simulink model "MainSim"  (R2024a)
settings: Solver=ode4  StartTime=0.0  StopTime=simtime  FixedStep=0.1  RelTol=1e-3
values from neighbouring files (symbols this model uses):
  C = [1 0 0 0 0 0 -1 0 0 0 0 0 ... (45 elements, 5x9)]    [C.mat]
undefined symbols (not defined in the file or in its folder): Ki, Kp, ssest, syys, utrim, xtrim
libraries: neural x680
(part 11 of 12)

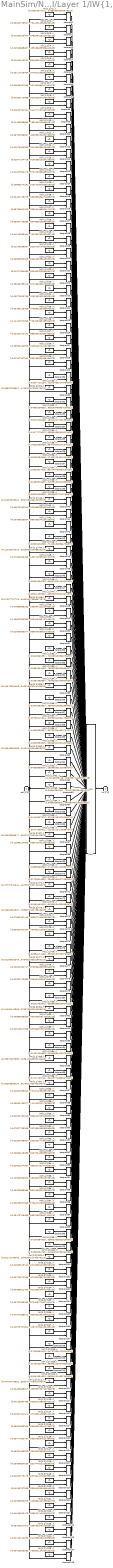
== system MainSim/NARX Neural Network PSI/Layer 1/IW{1,2} ==
  "pd{1,2}" : Inport  PortDimensions=5  SampleTime=0.1
      mask Display: e = 0.06;c1 = [120 230 180]/255;c2 = ([120 230 180]+0)/(256+128);c3 = ([120 230 180]+128)/(256+128);patch([0 1 1 0],[0 0 1 1],c1);patch([0 1 1 1-e 1-e 0+e],[0 0 1 1-e 0+e 0+e],c2);patch([0 0 1 1-e 0+e 0+e],[0 1 1 1-e 1-e 0+e],c3);plot([0 1 1 0 0],[0 0 1 1 0]);
  "IW{1,2}(1,:)'" : Constant  Value=[-0.036215741013831952155310744956295820884406566619873046875;5.60879432784090365695338353813070852993405424058437347412109375e-05;-0.0124726147008203773480783382865411113016307353973388671875;-0.022891343060553341615115385820899973623454570770263671875;0.0202316851446837260575239980653350357897579669952392578125]
      mask Display: e = 0.06;c1 = [120 150 230]/255;c2 = ([120 150 230]+0)/383;c3 = ([120 150 230]+128)/383;patch([0 1 1 0],[0 0 1 1],c1);patch([0 1 1 1-e 1-e 0+e],[0 0 1 1-e 0+e 0+e],c2);patch([0 0 1 1-e 0+e 0+e],[0 1 1 1-e 1-e 0+e],c3);plot([0 1 1 0 0],[0 0 1 1 0]);disp('Weights');
  "IW{1,2}(10,:)'" : Constant  Value=[0.0143353889361894325238377945197498775087296962738037109375;-0.007381001264767226253959986337349619134329259395599365234375;-0.027592123266478564558301656006733537651598453521728515625;0.12178092758731294542595691154929227195680141448974609375;0.1687882806982235195381036874096025712788105010986328125]
      mask Display: e = 0.06;c1 = [120 150 230]/255;c2 = ([120 150 230]+0)/383;c3 = ([120 150 230]+128)/383;patch([0 1 1 0],[0 0 1 1],c1);patch([0 1 1 1-e 1-e 0+e],[0 0 1 1-e 0+e 0+e],c2);patch([0 0 1 1-e 0+e 0+e],[0 1 1 1-e 1-e 0+e],c3);plot([0 1 1 0 0],[0 0 1 1 0]);disp('Weights');
  "IW{1,2}(100,:)'" : Constant  Value=[0.04365501765996560035176798919565044343471527099609375;0.00790203801594095180116372745260377996601164340972900390625;0.01233722257321183228551131350059222313575446605682373046875;-0.036139685759429558686850469939599861390888690948486328125;-0.07424116624505507078257693365230807103216648101806640625]
      mask Display: e = 0.06;c1 = [120 150 230]/255;c2 = ([120 150 230]+0)/383;c3 = ([120 150 230]+128)/383;patch([0 1 1 0],[0 0 1 1],c1);patch([0 1 1 1-e 1-e 0+e],[0 0 1 1-e 0+e 0+e],c2);patch([0 0 1 1-e 0+e 0+e],[0 1 1 1-e 1-e 0+e],c3);plot([0 1 1 0 0],[0 0 1 1 0]);disp('Weights');
  "IW{1,2}(101,:)'" : Constant  Value=[-0.021711480455671894329583437865949235856533050537109375;-0.00807230767060648606026074247665746952407062053680419921875;-0.0002256341632367506698508829998672808869741857051849365234375;-0.0262979277440466806259333765183328068815171718597412109375;-0.011795589954404724075676114125599269755184650421142578125]
      mask Display: e = 0.06;c1 = [120 150 230]/255;c2 = ([120 150 230]+0)/383;c3 = ([120 150 230]+128)/383;patch([0 1 1 0],[0 0 1 1],c1);patch([0 1 1 1-e 1-e 0+e],[0 0 1 1-e 0+e 0+e],c2);patch([0 0 1 1-e 0+e 0+e],[0 1 1 1-e 1-e 0+e],c3);plot([0 1 1 0 0],[0 0 1 1 0]);disp('Weights');
  "IW{1,2}(102,:)'" : Constant  Value=[-0.0190924914203203406615205750540553708560764789581298828125;-0.04084976908135444506608990877793985418975353240966796875;0.01049922442944002665132785523383063264191150665283203125;-0.09276854951829956175135549756305408664047718048095703125;-0.0969975545198410726843718521195114590227603912353515625]
      mask Display: e = 0.06;c1 = [120 150 230]/255;c2 = ([120 150 230]+0)/383;c3 = ([120 150 230]+128)/383;patch([0 1 1 0],[0 0 1 1],c1);patch([0 1 1 1-e 1-e 0+e],[0 0 1 1-e 0+e 0+e],c2);patch([0 0 1 1-e 0+e 0+e],[0 1 1 1-e 1-e 0+e],c3);plot([0 1 1 0 0],[0 0 1 1 0]);disp('Weights');
  "IW{1,2}(103,:)'" : Constant  Value=[-0.037290702881635669208026939713818137533962726593017578125;0.01315953443051502171068367630368811660446226596832275390625;-0.0152059084062875042586693297153033199720084667205810546875;0.011674382342164314751986609053346910513937473297119140625;0.05572879366650791699289158032115665264427661895751953125]
      mask Display: e = 0.06;c1 = [120 150 230]/255;c2 = ([120 150 230]+0)/383;c3 = ([120 150 230]+128)/383;patch([0 1 1 0],[0 0 1 1],c1);patch([0 1 1 1-e 1-e 0+e],[0 0 1 1-e 0+e 0+e],c2);patch([0 0 1 1-e 0+e 0+e],[0 1 1 1-e 1-e 0+e],c3);plot([0 1 1 0 0],[0 0 1 1 0]);disp('Weights');
  "IW{1,2}(104,:)'" : Constant  Value=[-0.00086611442030111451817475654024747200310230255126953125;0.00108653245732205617178622869545279172598384320735931396484375;-0.0300000825214495787929269710048174601979553699493408203125;-0.016134310882040293899652994014104478992521762847900390625;0.044166595105996526993141770844886195845901966094970703125]
      mask Display: e = 0.06;c1 = [120 150 230]/255;c2 = ([120 150 230]+0)/383;c3 = ([120 150 230]+128)/383;patch([0 1 1 0],[0 0 1 1],c1);patch([0 1 1 1-e 1-e 0+e],[0 0 1 1-e 0+e 0+e],c2);patch([0 0 1 1-e 0+e 0+e],[0 1 1 1-e 1-e 0+e],c3);plot([0 1 1 0 0],[0 0 1 1 0]);disp('Weights');
  "IW{1,2}(105,:)'" : Constant  Value=[-0.037679363331454086838423478411641553975641727447509765625;0.02462650060839417787139637994187069125473499298095703125;0.0258598451661068880202964948011867818422615528106689453125;0.06634544811163727018321623063457082025706768035888671875;0.0210341337753423944512132237605328555218875408172607421875]
      mask Display: e = 0.06;c1 = [120 150 230]/255;c2 = ([120 150 230]+0)/383;c3 = ([120 150 230]+128)/383;patch([0 1 1 0],[0 0 1 1],c1);patch([0 1 1 1-e 1-e 0+e],[0 0 1 1-e 0+e 0+e],c2);patch([0 0 1 1-e 0+e 0+e],[0 1 1 1-e 1-e 0+e],c3);plot([0 1 1 0 0],[0 0 1 1 0]);disp('Weights');
  "IW{1,2}(106,:)'" : Constant  Value=[-0.0797208552113842505715268771382397972047328948974609375;-0.004680836346071730151574552536430928739719092845916748046875;0.04106850000033028524892841915061580948531627655029296875;-0.020138888342617448923288492323990794830024242401123046875;-0.0637193215808195823068871277428115718066692352294921875]
      mask Display: e = 0.06;c1 = [120 150 230]/255;c2 = ([120 150 230]+0)/383;c3 = ([120 150 230]+128)/383;patch([0 1 1 0],[0 0 1 1],c1);patch([0 1 1 1-e 1-e 0+e],[0 0 1 1-e 0+e 0+e],c2);patch([0 0 1 1-e 0+e 0+e],[0 1 1 1-e 1-e 0+e],c3);plot([0 1 1 0 0],[0 0 1 1 0]);disp('Weights');
  "IW{1,2}(107,:)'" : Constant  Value=[-0.018787076045366134235958810450028977356851100921630859375;0.038027756628217591894358662329977960325777530670166015625;0.01064586703009156622157238558656899840570986270904541015625;0.043188689285246890936509345237936940975487232208251953125;0.0201443282352079984509618526544727501459419727325439453125]
      mask Display: e = 0.06;c1 = [120 150 230]/255;c2 = ([120 150 230]+0)/383;c3 = ([120 150 230]+128)/383;patch([0 1 1 0],[0 0 1 1],c1);patch([0 1 1 1-e 1-e 0+e],[0 0 1 1-e 0+e 0+e],c2);patch([0 0 1 1-e 0+e 0+e],[0 1 1 1-e 1-e 0+e],c3);plot([0 1 1 0 0],[0 0 1 1 0]);disp('Weights');
  "IW{1,2}(108,:)'" : Constant  Value=[0.07009550418119052384025025048686075024306774139404296875;0.0392247917688698655158674455378786660730838775634765625;-0.06753931344667206404519532725316821597516536712646484375;-0.131338914956515451226692903219372965395450592041015625;-0.01805059031289417414978260012503596954047679901123046875]
      mask Display: e = 0.06;c1 = [120 150 230]/255;c2 = ([120 150 230]+0)/383;c3 = ([120 150 230]+128)/383;patch([0 1 1 0],[0 0 1 1],c1);patch([0 1 1 1-e 1-e 0+e],[0 0 1 1-e 0+e 0+e],c2);patch([0 0 1 1-e 0+e 0+e],[0 1 1 1-e 1-e 0+e],c3);plot([0 1 1 0 0],[0 0 1 1 0]);disp('Weights');
  "IW{1,2}(109,:)'" : Constant  Value=[0.027903264592611394523391510347209987230598926544189453125;-0.018209312551109406441707250223771552555263042449951171875;-0.029560053340425600232332925543232704512774944305419921875;-0.058448597479059671844225931636174209415912628173828125;-0.004503732822406581078056309053181394119746983051300048828125]
      mask Display: e = 0.06;c1 = [120 150 230]/255;c2 = ([120 150 230]+0)/383;c3 = ([120 150 230]+128)/383;patch([0 1 1 0],[0 0 1 1],c1);patch([0 1 1 1-e 1-e 0+e],[0 0 1 1-e 0+e 0+e],c2);patch([0 0 1 1-e 0+e 0+e],[0 1 1 1-e 1-e 0+e],c3);plot([0 1 1 0 0],[0 0 1 1 0]);disp('Weights');
  "IW{1,2}(11,:)'" : Constant  Value=[-0.06784536567335834600367405755605432204902172088623046875;0.057055285864451001087704895553542883135378360748291015625;-0.002680767858079032874007996412046850309707224369049072265625;-0.00491724240786181772400187384164382820017635822296142578125;0.0203640435528099732198636928615087526850402355194091796875]
      mask Display: e = 0.06;c1 = [120 150 230]/255;c2 = ([120 150 230]+0)/383;c3 = ([120 150 230]+128)/383;patch([0 1 1 0],[0 0 1 1],c1);patch([0 1 1 1-e 1-e 0+e],[0 0 1 1-e 0+e 0+e],c2);patch([0 0 1 1-e 0+e 0+e],[0 1 1 1-e 1-e 0+e],c3);plot([0 1 1 0 0],[0 0 1 1 0]);disp('Weights');
  "IW{1,2}(110,:)'" : Constant  Value=[0.0343435492268395758941323947510682046413421630859375;0.01295666519578909069154715183458392857573926448822021484375;0.00708078622384187596205951109595844172872602939605712890625;0.033670595471844887158763270917916088365018367767333984375;0.0003231989567397515147363640242161864080117084085941314697265625]
      mask Display: e = 0.06;c1 = [120 150 230]/255;c2 = ([120 150 230]+0)/383;c3 = ([120 150 230]+128)/383;patch([0 1 1 0],[0 0 1 1],c1);patch([0 1 1 1-e 1-e 0+e],[0 0 1 1-e 0+e 0+e],c2);patch([0 0 1 1-e 0+e 0+e],[0 1 1 1-e 1-e 0+e],c3);plot([0 1 1 0 0],[0 0 1 1 0]);disp('Weights');
  "IW{1,2}(111,:)'" : Constant  Value=[-0.047944793321469260372058585062404745258390903472900390625;0.0476529114527805830459072922167251817882061004638671875;0.024448937097989863198588267323430045507848262786865234375;0.11063606950268144168969541851765825413167476654052734375;0.07017883922331434598529398272148682735860347747802734375]
      mask Display: e = 0.06;c1 = [120 150 230]/255;c2 = ([120 150 230]+0)/383;c3 = ([120 150 230]+128)/383;patch([0 1 1 0],[0 0 1 1],c1);patch([0 1 1 1-e 1-e 0+e],[0 0 1 1-e 0+e 0+e],c2);patch([0 0 1 1-e 0+e 0+e],[0 1 1 1-e 1-e 0+e],c3);plot([0 1 1 0 0],[0 0 1 1 0]);disp('Weights');
  "IW{1,2}(112,:)'" : Constant  Value=[-0.00433683917985687970853003747606635442934930324554443359375;-0.01179886612651101333859582354079975630156695842742919921875;0.038499504319846812594452245548382052220404148101806640625;0.0003384644029183101160244973026891557310591451823711395263671875;-0.07193478992266981453251872835608082823455333709716796875]
      mask Display: e = 0.06;c1 = [120 150 230]/255;c2 = ([120 150 230]+0)/383;c3 = ([120 150 230]+128)/383;patch([0 1 1 0],[0 0 1 1],c1);patch([0 1 1 1-e 1-e 0+e],[0 0 1 1-e 0+e 0+e],c2);patch([0 0 1 1-e 0+e 0+e],[0 1 1 1-e 1-e 0+e],c3);plot([0 1 1 0 0],[0 0 1 1 0]);disp('Weights');
  "IW{1,2}(113,:)'" : Constant  Value=[0.04126094495978659126844689808422117494046688079833984375;0.0715011784149503226704069902552873827517032623291015625;-0.029332417097580047726790297701882082037627696990966796875;0.044113255766767521526272588516803807578980922698974609375;0.0749107750095812374713233339207363314926624298095703125]
      mask Display: e = 0.06;c1 = [120 150 230]/255;c2 = ([120 150 230]+0)/383;c3 = ([120 150 230]+128)/383;patch([0 1 1 0],[0 0 1 1],c1);patch([0 1 1 1-e 1-e 0+e],[0 0 1 1-e 0+e 0+e],c2);patch([0 0 1 1-e 0+e 0+e],[0 1 1 1-e 1-e 0+e],c3);plot([0 1 1 0 0],[0 0 1 1 0]);disp('Weights');
  "IW{1,2}(114,:)'" : Constant  Value=[-0.0156722467499324051576348182379661011509597301483154296875;0.005390025467857165013263465169757182593457400798797607421875;-0.0265373292893429091332535563196870498359203338623046875;0.0001589057175574463335980535116931378070148639380931854248046875;0.056802380327879632704313195290524163283407688140869140625]
      mask Display: e = 0.06;c1 = [120 150 230]/255;c2 = ([120 150 230]+0)/383;c3 = ([120 150 230]+128)/383;patch([0 1 1 0],[0 0 1 1],c1);patch([0 1 1 1-e 1-e 0+e],[0 0 1 1-e 0+e 0+e],c2);patch([0 0 1 1-e 0+e 0+e],[0 1 1 1-e 1-e 0+e],c3);plot([0 1 1 0 0],[0 0 1 1 0]);disp('Weights');
  "IW{1,2}(115,:)'" : Constant  Value=[0.05524953329222011266796954487290349788963794708251953125;-0.006431394135198806143172145510789050604216754436492919921875;-0.062335716365556452511764717883124831132590770721435546875;-0.0139287598417728621102984476465280749835073947906494140625;0.08893091657780860526116839537280611693859100341796875]
      mask Display: e = 0.06;c1 = [120 150 230]/255;c2 = ([120 150 230]+0)/383;c3 = ([120 150 230]+128)/383;patch([0 1 1 0],[0 0 1 1],c1);patch([0 1 1 1-e 1-e 0+e],[0 0 1 1-e 0+e 0+e],c2);patch([0 0 1 1-e 0+e 0+e],[0 1 1 1-e 1-e 0+e],c3);plot([0 1 1 0 0],[0 0 1 1 0]);disp('Weights');
  "IW{1,2}(116,:)'" : Constant  Value=[-0.007770007347034535438723423794726841151714324951171875;0.00179730026795966242765534293113205421832390129566192626953125;-0.0180713848062352931689300561401978484354913234710693359375;-0.0309363499383004843246158799274780903942883014678955078125;0.0110713119878358932923756441368823288939893245697021484375]
      mask Display: e = 0.06;c1 = [120 150 230]/255;c2 = ([120 150 230]+0)/383;c3 = ([120 150 230]+128)/383;patch([0 1 1 0],[0 0 1 1],c1);patch([0 1 1 1-e 1-e 0+e],[0 0 1 1-e 0+e 0+e],c2);patch([0 0 1 1-e 0+e 0+e],[0 1 1 1-e 1-e 0+e],c3);plot([0 1 1 0 0],[0 0 1 1 0]);disp('Weights');
  "IW{1,2}(117,:)'" : Constant  Value=[0.05331469629343903171569962751163984648883342742919921875;-0.00788955748275679651093650335269558127038180828094482421875;-0.041513050258057897223817889198471675626933574676513671875;-0.0931362590739594764510655977574060671031475067138671875;-0.0248034327679624612417175200107521959580481052398681640625]
      mask Display: e = 0.06;c1 = [120 150 230]/255;c2 = ([120 150 230]+0)/383;c3 = ([120 150 230]+128)/383;patch([0 1 1 0],[0 0 1 1],c1);patch([0 1 1 1-e 1-e 0+e],[0 0 1 1-e 0+e 0+e],c2);patch([0 0 1 1-e 0+e 0+e],[0 1 1 1-e 1-e 0+e],c3);plot([0 1 1 0 0],[0 0 1 1 0]);disp('Weights');
  "IW{1,2}(118,:)'" : Constant  Value=[-0.03436657036450664615134797941209399141371250152587890625;-0.0019304738179542059277327137323254646616987884044647216796875;-0.0004147806349897751264886591737734988782904110848903656005859375;-0.05308334180004233016081371943073463626205921173095703125;-0.031944155710130116287981394407324842177331447601318359375]
      mask Display: e = 0.06;c1 = [120 150 230]/255;c2 = ([120 150 230]+0)/383;c3 = ([120 150 230]+128)/383;patch([0 1 1 0],[0 0 1 1],c1);patch([0 1 1 1-e 1-e 0+e],[0 0 1 1-e 0+e 0+e],c2);patch([0 0 1 1-e 0+e 0+e],[0 1 1 1-e 1-e 0+e],c3);plot([0 1 1 0 0],[0 0 1 1 0]);disp('Weights');
  "IW{1,2}(119,:)'" : Constant  Value=[-0.0194977917569244089956992382894895854406058788299560546875;-0.004678634104345880985464933843331891694106161594390869140625;0.05001953115971992380739408190493122674524784088134765625;-0.051358167481461831915812155102685210295021533966064453125;-0.1383571964667627274270245152365532703697681427001953125]
      mask Display: e = 0.06;c1 = [120 150 230]/255;c2 = ([120 150 230]+0)/383;c3 = ([120 150 230]+128)/383;patch([0 1 1 0],[0 0 1 1],c1);patch([0 1 1 1-e 1-e 0+e],[0 0 1 1-e 0+e 0+e],c2);patch([0 0 1 1-e 0+e 0+e],[0 1 1 1-e 1-e 0+e],c3);plot([0 1 1 0 0],[0 0 1 1 0]);disp('Weights');
  "IW{1,2}(12,:)'" : Constant  Value=[-0.016753003332310056894272065619588829576969146728515625;0.0285850979291362959633371332301976508460938930511474609375;0.01179355362913673925528978969623494776897132396697998046875;0.050343408315679884224014273286229581572115421295166015625;0.0247000745497743222356401560091399005614221096038818359375]
      mask Display: e = 0.06;c1 = [120 150 230]/255;c2 = ([120 150 230]+0)/383;c3 = ([120 150 230]+128)/383;patch([0 1 1 0],[0 0 1 1],c1);patch([0 1 1 1-e 1-e 0+e],[0 0 1 1-e 0+e 0+e],c2);patch([0 0 1 1-e 0+e 0+e],[0 1 1 1-e 1-e 0+e],c3);plot([0 1 1 0 0],[0 0 1 1 0]);disp('Weights');
  "IW{1,2}(120,:)'" : Constant  Value=[0.04108767993558308517787480695915292017161846160888671875;0.039495322133149012022723667314494377933442592620849609375;-0.0567553029714990275866881574984290637075901031494140625;-0.0734544757114203861192436306737363338470458984375;0.024152857690850494665202319310992606915533542633056640625]
      mask Display: e = 0.06;c1 = [120 150 230]/255;c2 = ([120 150 230]+0)/383;c3 = ([120 150 230]+128)/383;patch([0 1 1 0],[0 0 1 1],c1);patch([0 1 1 1-e 1-e 0+e],[0 0 1 1-e 0+e 0+e],c2);patch([0 0 1 1-e 0+e 0+e],[0 1 1 1-e 1-e 0+e],c3);plot([0 1 1 0 0],[0 0 1 1 0]);disp('Weights');
  "IW{1,2}(121,:)'" : Constant  Value=[-0.0025880937315550388462537245715111566823907196521759033203125;0.039533967041615707127544254717577132396399974822998046875;-0.0297957396708810710872494809109412017278373241424560546875;0.0175000063548198976637326751415457692928612232208251953125;0.07581829281669293096879158611045568250119686126708984375]
      mask Display: e = 0.06;c1 = [120 150 230]/255;c2 = ([120 150 230]+0)/383;c3 = ([120 150 230]+128)/383;patch([0 1 1 0],[0 0 1 1],c1);patch([0 1 1 1-e 1-e 0+e],[0 0 1 1-e 0+e 0+e],c2);patch([0 0 1 1-e 0+e 0+e],[0 1 1 1-e 1-e 0+e],c3);plot([0 1 1 0 0],[0 0 1 1 0]);disp('Weights');
  "IW{1,2}(122,:)'" : Constant  Value=[-0.040482004756239274578799580694976611994206905364990234375;-0.0084828557419303167452806491155570256523787975311279296875;0.0373609757745712867116338884443393908441066741943359375;0.066359503360522709147772957294364459812641143798828125;0.002060270763875653166063983690037275664508342742919921875]
      mask Display: e = 0.06;c1 = [120 150 230]/255;c2 = ([120 150 230]+0)/383;c3 = ([120 150 230]+128)/383;patch([0 1 1 0],[0 0 1 1],c1);patch([0 1 1 1-e 1-e 0+e],[0 0 1 1-e 0+e 0+e],c2);patch([0 0 1 1-e 0+e 0+e],[0 1 1 1-e 1-e 0+e],c3);plot([0 1 1 0 0],[0 0 1 1 0]);disp('Weights');
  "IW{1,2}(123,:)'" : Constant  Value=[0.03416517870281386703990023079313687048852443695068359375;-0.01497263813686294277316424228274627239443361759185791015625;-0.03330456176119432620819083012975170277059078216552734375;-0.037996513495981439068049922980208066292107105255126953125;0.020667609928990589296393665108553250320255756378173828125]
      mask Display: e = 0.06;c1 = [120 150 230]/255;c2 = ([120 150 230]+0)/383;c3 = ([120 150 230]+128)/383;patch([0 1 1 0],[0 0 1 1],c1);patch([0 1 1 1-e 1-e 0+e],[0 0 1 1-e 0+e 0+e],c2);patch([0 0 1 1-e 0+e 0+e],[0 1 1 1-e 1-e 0+e],c3);plot([0 1 1 0 0],[0 0 1 1 0]);disp('Weights');
  "IW{1,2}(124,:)'" : Constant  Value=[-0.0474311025689617971057288059455459006130695343017578125;-0.0084990343063844515925087108598745544441044330596923828125;0.026522056192171482302821772236711694858968257904052734375;-0.044803604650022366140404983525513671338558197021484375;-0.0706294569851905473800712798038148321211338043212890625]
      mask Display: e = 0.06;c1 = [120 150 230]/255;c2 = ([120 150 230]+0)/383;c3 = ([120 150 230]+128)/383;patch([0 1 1 0],[0 0 1 1],c1);patch([0 1 1 1-e 1-e 0+e],[0 0 1 1-e 0+e 0+e],c2);patch([0 0 1 1-e 0+e 0+e],[0 1 1 1-e 1-e 0+e],c3);plot([0 1 1 0 0],[0 0 1 1 0]);disp('Weights');
  "IW{1,2}(125,:)'" : Constant  Value=[-0.0041352633313304666684562249656664789654314517974853515625;-0.05883224234928326190630087921817903406918048858642578125;0.0446078165266844128833412241874611936509609222412109375;0.10478718971399607340355686346811125986278057098388671875;0.0148238784771977834264777840189708513207733631134033203125]
      mask Display: e = 0.06;c1 = [120 150 230]/255;c2 = ([120 150 230]+0)/383;c3 = ([120 150 230]+128)/383;patch([0 1 1 0],[0 0 1 1],c1);patch([0 1 1 1-e 1-e 0+e],[0 0 1 1-e 0+e 0+e],c2);patch([0 0 1 1-e 0+e 0+e],[0 1 1 1-e 1-e 0+e],c3);plot([0 1 1 0 0],[0 0 1 1 0]);disp('Weights');
  "IW{1,2}(13,:)'" : Constant  Value=[0.02877144728087617508993645287773688323795795440673828125;-0.00416256033542508098455048326513860956765711307525634765625;-0.05354133524824943035635982369058183394372463226318359375;0.06915665582352735485383021796224056743085384368896484375;0.1594088150118338764738012969246483407914638519287109375]
      mask Display: e = 0.06;c1 = [120 150 230]/255;c2 = ([120 150 230]+0)/383;c3 = ([120 150 230]+128)/383;patch([0 1 1 0],[0 0 1 1],c1);patch([0 1 1 1-e 1-e 0+e],[0 0 1 1-e 0+e 0+e],c2);patch([0 0 1 1-e 0+e 0+e],[0 1 1 1-e 1-e 0+e],c3);plot([0 1 1 0 0],[0 0 1 1 0]);disp('Weights');
  "IW{1,2}(14,:)'" : Constant  Value=[-0.04207822478421353873390131639098399318754673004150390625;-0.01012660696863064424544376151970936916768550872802734375;-0.0159495140224796549954788815739448182284832000732421875;0.07987577448249101597088639437060919590294361114501953125;0.12227185354109675052836081476925755850970745086669921875]
      mask Display: e = 0.06;c1 = [120 150 230]/255;c2 = ([120 150 230]+0)/383;c3 = ([120 150 230]+128)/383;patch([0 1 1 0],[0 0 1 1],c1);patch([0 1 1 1-e 1-e 0+e],[0 0 1 1-e 0+e 0+e],c2);patch([0 0 1 1-e 0+e 0+e],[0 1 1 1-e 1-e 0+e],c3);plot([0 1 1 0 0],[0 0 1 1 0]);disp('Weights');
  "IW{1,2}(15,:)'" : Constant  Value=[0.29869274291982061964034755874308757483959197998046875;-0.01021093824654447333732942837514201528392732143402099609375;-0.133787597215125175775796151356189511716365814208984375;-0.172595542507849974978029194971895776689052581787109375;-0.02052316749456706279630680000991560518741607666015625]
      mask Display: e = 0.06;c1 = [120 150 230]/255;c2 = ([120 150 230]+0)/383;c3 = ([120 150 230]+128)/383;patch([0 1 1 0],[0 0 1 1],c1);patch([0 1 1 1-e 1-e 0+e],[0 0 1 1-e 0+e 0+e],c2);patch([0 0 1 1-e 0+e 0+e],[0 1 1 1-e 1-e 0+e],c3);plot([0 1 1 0 0],[0 0 1 1 0]);disp('Weights');
  "IW{1,2}(16,:)'" : Constant  Value=[-0.024547451758043216385463125561727792955935001373291015625;0.0242133921509202522381887234814712428487837314605712890625;-0.0264493059226358594171468752165310434065759181976318359375;-0.0185513623748869392604543548941364861093461513519287109375;0.04532930063992067493128246269407100044190883636474609375]
      mask Display: e = 0.06;c1 = [120 150 230]/255;c2 = ([120 150 230]+0)/383;c3 = ([120 150 230]+128)/383;patch([0 1 1 0],[0 0 1 1],c1);patch([0 1 1 1-e 1-e 0+e],[0 0 1 1-e 0+e 0+e],c2);patch([0 0 1 1-e 0+e 0+e],[0 1 1 1-e 1-e 0+e],c3);plot([0 1 1 0 0],[0 0 1 1 0]);disp('Weights');
  "IW{1,2}(17,:)'" : Constant  Value=[0.05795842020262510774220032772063859738409519195556640625;-0.047212472629454112216240702082359348423779010772705078125;-0.01400780075910705406438960807236071559600532054901123046875;0.08021370444535895483095799818329396657645702362060546875;0.08029121187727565611691460389920393936336040496826171875]
      mask Display: e = 0.06;c1 = [120 150 230]/255;c2 = ([120 150 230]+0)/383;c3 = ([120 150 230]+128)/383;patch([0 1 1 0],[0 0 1 1],c1);patch([0 1 1 1-e 1-e 0+e],[0 0 1 1-e 0+e 0+e],c2);patch([0 0 1 1-e 0+e 0+e],[0 1 1 1-e 1-e 0+e],c3);plot([0 1 1 0 0],[0 0 1 1 0]);disp('Weights');
  "IW{1,2}(18,:)'" : Constant  Value=[-0.0500471888622528171541858910131850279867649078369140625;0.006787486156340967642652817204407256213016808032989501953125;0.053674233914009487900198536181051167659461498260498046875;0.03963848185398781420740732528429361991584300994873046875;-0.0503718037103643434537758594160550273954868316650390625]
      mask Display: e = 0.06;c1 = [120 150 230]/255;c2 = ([120 150 230]+0)/383;c3 = ([120 150 230]+128)/383;patch([0 1 1 0],[0 0 1 1],c1);patch([0 1 1 1-e 1-e 0+e],[0 0 1 1-e 0+e 0+e],c2);patch([0 0 1 1-e 0+e 0+e],[0 1 1 1-e 1-e 0+e],c3);plot([0 1 1 0 0],[0 0 1 1 0]);disp('Weights');
  "IW{1,2}(19,:)'" : Constant  Value=[-0.041135350040979512531436057543032802641391754150390625;0.005798917039239792625693326044711284339427947998046875;-0.01070238640528972141885422075802125618793070316314697265625;-0.0001734097151971002929819742899297807525726966559886932373046875;0.0385962924509451188459507875450071878731250762939453125]
      mask Display: e = 0.06;c1 = [120 150 230]/255;c2 = ([120 150 230]+0)/383;c3 = ([120 150 230]+128)/383;patch([0 1 1 0],[0 0 1 1],c1);patch([0 1 1 1-e 1-e 0+e],[0 0 1 1-e 0+e 0+e],c2);patch([0 0 1 1-e 0+e 0+e],[0 1 1 1-e 1-e 0+e],c3);plot([0 1 1 0 0],[0 0 1 1 0]);disp('Weights');
  "IW{1,2}(2,:)'" : Constant  Value=[-0.0304971550741986729970989244975498877465724945068359375;0.00192189419500140841294555382745556926238350570201873779296875;-0.0179367529279445027390327283001170144416391849517822265625;0.019356188507245401797529638088235515169799327850341796875;0.0644836077260156070867225253095966763794422149658203125]
      mask Display: e = 0.06;c1 = [120 150 230]/255;c2 = ([120 150 230]+0)/383;c3 = ([120 150 230]+128)/383;patch([0 1 1 0],[0 0 1 1],c1);patch([0 1 1 1-e 1-e 0+e],[0 0 1 1-e 0+e 0+e],c2);patch([0 0 1 1-e 0+e 0+e],[0 1 1 1-e 1-e 0+e],c3);plot([0 1 1 0 0],[0 0 1 1 0]);disp('Weights');
  "IW{1,2}(20,:)'" : Constant  Value=[0.01249098007626906793599008693718133145011961460113525390625;-0.007201876217956033714162611403253322350792586803436279296875;0.016084658684607712475500562732122489251196384429931640625;0.04125399740179515328808435015162103809416294097900390625;0.002089202347441310170239603394293226301670074462890625]
      mask Display: e = 0.06;c1 = [120 150 230]/255;c2 = ([120 150 230]+0)/383;c3 = ([120 150 230]+128)/383;patch([0 1 1 0],[0 0 1 1],c1);patch([0 1 1 1-e 1-e 0+e],[0 0 1 1-e 0+e 0+e],c2);patch([0 0 1 1-e 0+e 0+e],[0 1 1 1-e 1-e 0+e],c3);plot([0 1 1 0 0],[0 0 1 1 0]);disp('Weights');
  "IW{1,2}(21,:)'" : Constant  Value=[-0.06392851645465306986704234759599785320460796356201171875;0.0160388436570271901426831817616402986459434032440185546875;0.002192562003192555057651258465512000839225947856903076171875;0.0199696660171350300061465787848646868951618671417236328125;0.038725099380477488730800672556142671965062618255615234375]
      mask Display: e = 0.06;c1 = [120 150 230]/255;c2 = ([120 150 230]+0)/383;c3 = ([120 150 230]+128)/383;patch([0 1 1 0],[0 0 1 1],c1);patch([0 1 1 1-e 1-e 0+e],[0 0 1 1-e 0+e 0+e],c2);patch([0 0 1 1-e 0+e 0+e],[0 1 1 1-e 1-e 0+e],c3);plot([0 1 1 0 0],[0 0 1 1 0]);disp('Weights');
  "IW{1,2}(22,:)'" : Constant  Value=[0.012276845552893787816284287828239030204713344573974609375;0.0088151271711112803852739006060801330022513866424560546875;0.007598114082104707144027511134254382341168820858001708984375;0.0391047021000519856581689737140550278127193450927734375;0.0137905173576384175448961144638815312646329402923583984375]
      mask Display: e = 0.06;c1 = [120 150 230]/255;c2 = ([120 150 230]+0)/383;c3 = ([120 150 230]+128)/383;patch([0 1 1 0],[0 0 1 1],c1);patch([0 1 1 1-e 1-e 0+e],[0 0 1 1-e 0+e 0+e],c2);patch([0 0 1 1-e 0+e 0+e],[0 1 1 1-e 1-e 0+e],c3);plot([0 1 1 0 0],[0 0 1 1 0]);disp('Weights');
  "IW{1,2}(23,:)'" : Constant  Value=[-0.051604951162480483528582908547832630574703216552734375;0.007319954958719951561285643748533402686007320880889892578125;0.062493991229892360828035435815763776190578937530517578125;0.000800132768911692403290825126305207959376275539398193359375;-0.1028039922590014143555237069449503906071186065673828125]
      mask Display: e = 0.06;c1 = [120 150 230]/255;c2 = ([120 150 230]+0)/383;c3 = ([120 150 230]+128)/383;patch([0 1 1 0],[0 0 1 1],c1);patch([0 1 1 1-e 1-e 0+e],[0 0 1 1-e 0+e 0+e],c2);patch([0 0 1 1-e 0+e 0+e],[0 1 1 1-e 1-e 0+e],c3);plot([0 1 1 0 0],[0 0 1 1 0]);disp('Weights');
  "IW{1,2}(24,:)'" : Constant  Value=[-0.032793297385889978723394477810870739631354808807373046875;-0.00725740186413058319114810501559986732900142669677734375;-0.01482374506319721584046700257886186591349542140960693359375;0.01783897550415276811452969241145183332264423370361328125;0.05849075686830969289520254505987395532429218292236328125]
      mask Display: e = 0.06;c1 = [120 150 230]/255;c2 = ([120 150 230]+0)/383;c3 = ([120 150 230]+128)/383;patch([0 1 1 0],[0 0 1 1],c1);patch([0 1 1 1-e 1-e 0+e],[0 0 1 1-e 0+e 0+e],c2);patch([0 0 1 1-e 0+e 0+e],[0 1 1 1-e 1-e 0+e],c3);plot([0 1 1 0 0],[0 0 1 1 0]);disp('Weights');
  "IW{1,2}(25,:)'" : Constant  Value=[-0.06493125428127856368920589602566906251013278961181640625;0.019983209331549518783521790510349092073738574981689453125;0.006643269015488183042161818292470343294553458690643310546875;-0.025892339937117224424323325138175277970731258392333984375;-0.01008616080997910315064647335248082526959478855133056640625]
      mask Display: e = 0.06;c1 = [120 150 230]/255;c2 = ([120 150 230]+0)/383;c3 = ([120 150 230]+128)/383;patch([0 1 1 0],[0 0 1 1],c1);patch([0 1 1 1-e 1-e 0+e],[0 0 1 1-e 0+e 0+e],c2);patch([0 0 1 1-e 0+e 0+e],[0 1 1 1-e 1-e 0+e],c3);plot([0 1 1 0 0],[0 0 1 1 0]);disp('Weights');
  "IW{1,2}(26,:)'" : Constant  Value=[-0.11411371366166600527236596462898887693881988525390625;-0.014919952910250604272146546236399444751441478729248046875;0.035183550637835125929342439121683128178119659423828125;0.049229100632018983618731766682685702107846736907958984375;0.025027472832522372481189876225471380166709423065185546875]
      mask Display: e = 0.06;c1 = [120 150 230]/255;c2 = ([120 150 230]+0)/383;c3 = ([120 150 230]+128)/383;patch([0 1 1 0],[0 0 1 1],c1);patch([0 1 1 1-e 1-e 0+e],[0 0 1 1-e 0+e 0+e],c2);patch([0 0 1 1-e 0+e 0+e],[0 1 1 1-e 1-e 0+e],c3);plot([0 1 1 0 0],[0 0 1 1 0]);disp('Weights');
  "IW{1,2}(27,:)'" : Constant  Value=[-0.0225197214182231535140044087484056944958865642547607421875;0.00736212559279472537887567540337840910069644451141357421875;-0.0135482223952490023199946023169104591943323612213134765625;0.1267734479519667945002225906137027777731418609619140625;0.1598281197241532558539489627946750260889530181884765625]
      mask Display: e = 0.06;c1 = [120 150 230]/255;c2 = ([120 150 230]+0)/383;c3 = ([120 150 230]+128)/383;patch([0 1 1 0],[0 0 1 1],c1);patch([0 1 1 1-e 1-e 0+e],[0 0 1 1-e 0+e 0+e],c2);patch([0 0 1 1-e 0+e 0+e],[0 1 1 1-e 1-e 0+e],c3);plot([0 1 1 0 0],[0 0 1 1 0]);disp('Weights');
  "IW{1,2}(28,:)'" : Constant  Value=[-0.059311625138291905467990972056213649921119213104248046875;-0.006290301789353855595188225180436347727663815021514892578125;0.06314302097769626531675868363890913315117359161376953125;0.05344895511540058430366428865454508922994136810302734375;-0.050575376419835442465267050238253432326018810272216796875]
      mask Display: e = 0.06;c1 = [120 150 230]/255;c2 = ([120 150 230]+0)/383;c3 = ([120 150 230]+128)/383;patch([0 1 1 0],[0 0 1 1],c1);patch([0 1 1 1-e 1-e 0+e],[0 0 1 1-e 0+e 0+e],c2);patch([0 0 1 1-e 0+e 0+e],[0 1 1 1-e 1-e 0+e],c3);plot([0 1 1 0 0],[0 0 1 1 0]);disp('Weights');
  "IW{1,2}(29,:)'" : Constant  Value=[-0.01257287940708441513482096496545636910013854503631591796875;-0.060395065174104041461067282625663210637867450714111328125;0.0491410156741179660055962585829547606408596038818359375;0.11318454423228278826751846963816205970942974090576171875;0.0175407405373560441874669635353711782954633235931396484375]
      mask Display: e = 0.06;c1 = [120 150 230]/255;c2 = ([120 150 230]+0)/383;c3 = ([120 150 230]+128)/383;patch([0 1 1 0],[0 0 1 1],c1);patch([0 1 1 1-e 1-e 0+e],[0 0 1 1-e 0+e 0+e],c2);patch([0 0 1 1-e 0+e 0+e],[0 1 1 1-e 1-e 0+e],c3);plot([0 1 1 0 0],[0 0 1 1 0]);disp('Weights');
  "IW{1,2}(3,:)'" : Constant  Value=[0.01309313474397146882799436440336648956872522830963134765625;-0.0023624846087443381222048532919188801315613090991973876953125;0.03366308921187970149002666175874765031039714813232421875;-0.059173336864796997891513541389940655790269374847412109375;-0.1257206456891222234872884655487723648548126220703125]
      mask Display: e = 0.06;c1 = [120 150 230]/255;c2 = ([120 150 230]+0)/383;c3 = ([120 150 230]+128)/383;patch([0 1 1 0],[0 0 1 1],c1);patch([0 1 1 1-e 1-e 0+e],[0 0 1 1-e 0+e 0+e],c2);patch([0 0 1 1-e 0+e 0+e],[0 1 1 1-e 1-e 0+e],c3);plot([0 1 1 0 0],[0 0 1 1 0]);disp('Weights');
  "IW{1,2}(30,:)'" : Constant  Value=[0.025477231045648675300530072718174778856337070465087890625;-0.00135394366011830683503569527914578429772518575191497802734375;-0.040717708986710905716410735522003960795700550079345703125;-0.03701740728450107764668786103356978856027126312255859375;0.036020242659014455044452773790908395312726497650146484375]
      mask Display: e = 0.06;c1 = [120 150 230]/255;c2 = ([120 150 230]+0)/383;c3 = ([120 150 230]+128)/383;patch([0 1 1 0],[0 0 1 1],c1);patch([0 1 1 1-e 1-e 0+e],[0 0 1 1-e 0+e 0+e],c2);patch([0 0 1 1-e 0+e 0+e],[0 1 1 1-e 1-e 0+e],c3);plot([0 1 1 0 0],[0 0 1 1 0]);disp('Weights');
  "IW{1,2}(31,:)'" : Constant  Value=[-0.08625788597820278902350565886081312783062458038330078125;-0.0015945059916173472298883684317161169019527733325958251953125;0.06342476053783045741862878230676869861781597137451171875;0.10024105858617382569519804746960289776325225830078125;0.0012201089509853405186412533822704062913544476032257080078125]
      mask Display: e = 0.06;c1 = [120 150 230]/255;c2 = ([120 150 230]+0)/383;c3 = ([120 150 230]+128)/383;patch([0 1 1 0],[0 0 1 1],c1);patch([0 1 1 1-e 1-e 0+e],[0 0 1 1-e 0+e 0+e],c2);patch([0 0 1 1-e 0+e 0+e],[0 1 1 1-e 1-e 0+e],c3);plot([0 1 1 0 0],[0 0 1 1 0]);disp('Weights');
  "IW{1,2}(32,:)'" : Constant  Value=[0.0493619805559266655592409733799286186695098876953125;-0.00868653048562638939456004294470403692685067653656005859375;-0.035731840462856878648523206720710732042789459228515625;-0.0809734967866642951772604419602430425584316253662109375;-0.0214995958189504211832687730066027143038809299468994140625]
      mask Display: e = 0.06;c1 = [120 150 230]/255;c2 = ([120 150 230]+0)/383;c3 = ([120 150 230]+128)/383;patch([0 1 1 0],[0 0 1 1],c1);patch([0 1 1 1-e 1-e 0+e],[0 0 1 1-e 0+e 0+e],c2);patch([0 0 1 1-e 0+e 0+e],[0 1 1 1-e 1-e 0+e],c3);plot([0 1 1 0 0],[0 0 1 1 0]);disp('Weights');
  "IW{1,2}(33,:)'" : Constant  Value=[0.00078708469671469002450214791366533972905017435550689697265625;0.01290650907813450411210087764857235015369951725006103515625;0.00046733306145279652522861457697445075609721243381500244140625;0.0818371342885702290903537914346088655292987823486328125;0.07175979228144686861146084311258164234459400177001953125]
      mask Display: e = 0.06;c1 = [120 150 230]/255;c2 = ([120 150 230]+0)/383;c3 = ([120 150 230]+128)/383;patch([0 1 1 0],[0 0 1 1],c1);patch([0 1 1 1-e 1-e 0+e],[0 0 1 1-e 0+e 0+e],c2);patch([0 0 1 1-e 0+e 0+e],[0 1 1 1-e 1-e 0+e],c3);plot([0 1 1 0 0],[0 0 1 1 0]);disp('Weights');
  "IW{1,2}(34,:)'" : Constant  Value=[0.01077275611740714615638392359642239171080291271209716796875;0.00133028746734454423293614322432176777510903775691986083984375;0.0193664306433864973067127124295438989065587520599365234375;0.0107677450955577201641144569066455005668103694915771484375;-0.03386511258580039707144493377199978567659854888916015625]
      mask Display: e = 0.06;c1 = [120 150 230]/255;c2 = ([120 150 230]+0)/383;c3 = ([120 150 230]+128)/383;patch([0 1 1 0],[0 0 1 1],c1);patch([0 1 1 1-e 1-e 0+e],[0 0 1 1-e 0+e 0+e],c2);patch([0 0 1 1-e 0+e 0+e],[0 1 1 1-e 1-e 0+e],c3);plot([0 1 1 0 0],[0 0 1 1 0]);disp('Weights');
  "IW{1,2}(35,:)'" : Constant  Value=[0.18620395058868377535787885790341533720493316650390625;0.0100748286496789123123374309898281353525817394256591796875;-0.098879894409355795215077478133025579154491424560546875;0.01040440551175022231011890738727743155322968959808349609375;0.12380432651178514824596987864424590952694416046142578125]
      mask Display: e = 0.06;c1 = [120 150 230]/255;c2 = ([120 150 230]+0)/383;c3 = ([120 150 230]+128)/383;patch([0 1 1 0],[0 0 1 1],c1);patch([0 1 1 1-e 1-e 0+e],[0 0 1 1-e 0+e 0+e],c2);patch([0 0 1 1-e 0+e 0+e],[0 1 1 1-e 1-e 0+e],c3);plot([0 1 1 0 0],[0 0 1 1 0]);disp('Weights');
  "IW{1,2}(36,:)'" : Constant  Value=[0.06283953308953653393853500119803356938064098358154296875;0.0474044244517978496933352516862214542925357818603515625;-0.03715211937521491203373358302997075952589511871337890625;0.04415491226897565180120608374636503867805004119873046875;0.08324477202418791021987232170431525446474552154541015625]
      mask Display: e = 0.06;c1 = [120 150 230]/255;c2 = ([120 150 230]+0)/383;c3 = ([120 150 230]+128)/383;patch([0 1 1 0],[0 0 1 1],c1);patch([0 1 1 1-e 1-e 0+e],[0 0 1 1-e 0+e 0+e],c2);patch([0 0 1 1-e 0+e 0+e],[0 1 1 1-e 1-e 0+e],c3);plot([0 1 1 0 0],[0 0 1 1 0]);disp('Weights');
  "IW{1,2}(37,:)'" : Constant  Value=[0.10920917616693780194392360272104269824922084808349609375;0.01126622469845997391579839330688628251664340496063232421875;-0.044533761331762129753730761194674414582550525665283203125;-0.0083748004414670833284173312449638615362346172332763671875;0.03457622051458771050835849791837972588837146759033203125]
      mask Display: e = 0.06;c1 = [120 150 230]/255;c2 = ([120 150 230]+0)/383;c3 = ([120 150 230]+128)/383;patch([0 1 1 0],[0 0 1 1],c1);patch([0 1 1 1-e 1-e 0+e],[0 0 1 1-e 0+e 0+e],c2);patch([0 0 1 1-e 0+e 0+e],[0 1 1 1-e 1-e 0+e],c3);plot([0 1 1 0 0],[0 0 1 1 0]);disp('Weights');
  "IW{1,2}(38,:)'" : Constant  Value=[0.01695513639634894931251807292937883175909519195556640625;-0.0025330445163571509679945048532090368098579347133636474609375;-0.040758353940759599332022133921782369725406169891357421875;-0.0020925452959782132010546629174996269284747540950775146484375;0.07235713108715287333883026121839066036045551300048828125]
      mask Display: e = 0.06;c1 = [120 150 230]/255;c2 = ([120 150 230]+0)/383;c3 = ([120 150 230]+128)/383;patch([0 1 1 0],[0 0 1 1],c1);patch([0 1 1 1-e 1-e 0+e],[0 0 1 1-e 0+e 0+e],c2);patch([0 0 1 1-e 0+e 0+e],[0 1 1 1-e 1-e 0+e],c3);plot([0 1 1 0 0],[0 0 1 1 0]);disp('Weights');
  "IW{1,2}(39,:)'" : Constant  Value=[0.060261089685000261695346779333704034797847270965576171875;0.0044640814274999503219465424308509682305157184600830078125;-0.00603114614744149069025525022880174219608306884765625;0.0174924484983870233423264295424814918078482151031494140625;0.00127217357190927550340819873753162028151564300060272216796875]
      mask Display: e = 0.06;c1 = [120 150 230]/255;c2 = ([120 150 230]+0)/383;c3 = ([120 150 230]+128)/383;patch([0 1 1 0],[0 0 1 1],c1);patch([0 1 1 1-e 1-e 0+e],[0 0 1 1-e 0+e 0+e],c2);patch([0 0 1 1-e 0+e 0+e],[0 1 1 1-e 1-e 0+e],c3);plot([0 1 1 0 0],[0 0 1 1 0]);disp('Weights');
  "IW{1,2}(4,:)'" : Constant  Value=[-0.019186886575522539566396318377883289940655231475830078125;-0.004502997689330270718321980183418418164364993572235107421875;0.04010690462661066491012462620346923358738422393798828125;0.03718928157781874188625437227528891526162624359130859375;-0.03608929516841043183550397088765748776495456695556640625]
      mask Display: e = 0.06;c1 = [120 150 230]/255;c2 = ([120 150 230]+0)/383;c3 = ([120 150 230]+128)/383;patch([0 1 1 0],[0 0 1 1],c1);patch([0 1 1 1-e 1-e 0+e],[0 0 1 1-e 0+e 0+e],c2);patch([0 0 1 1-e 0+e 0+e],[0 1 1 1-e 1-e 0+e],c3);plot([0 1 1 0 0],[0 0 1 1 0]);disp('Weights');
  "IW{1,2}(40,:)'" : Constant  Value=[-0.01251919004518711568685329638128678197972476482391357421875;-0.0074290693420022320403450777348552946932613849639892578125;-0.00477620600851305469880525578219021554104983806610107421875;-0.07286144105941876059073791793707641772925853729248046875;-0.0505689571929537340366778153111226856708526611328125]
      mask Display: e = 0.06;c1 = [120 150 230]/255;c2 = ([120 150 230]+0)/383;c3 = ([120 150 230]+128)/383;patch([0 1 1 0],[0 0 1 1],c1);patch([0 1 1 1-e 1-e 0+e],[0 0 1 1-e 0+e 0+e],c2);patch([0 0 1 1-e 0+e 0+e],[0 1 1 1-e 1-e 0+e],c3);plot([0 1 1 0 0],[0 0 1 1 0]);disp('Weights');
  "IW{1,2}(41,:)'" : Constant  Value=[-0.00973192340427684286774390187702010734938085079193115234375;-0.00828568828601327321548009052776251337490975856781005859375;-0.03291887610818965137493563588577671907842159271240234375;0.02531277885914863523542095435914234258234500885009765625;0.0907027874736728023652432284507085569202899932861328125]
      mask Display: e = 0.06;c1 = [120 150 230]/255;c2 = ([120 150 230]+0)/383;c3 = ([120 150 230]+128)/383;patch([0 1 1 0],[0 0 1 1],c1);patch([0 1 1 1-e 1-e 0+e],[0 0 1 1-e 0+e 0+e],c2);patch([0 0 1 1-e 0+e 0+e],[0 1 1 1-e 1-e 0+e],c3);plot([0 1 1 0 0],[0 0 1 1 0]);disp('Weights');
  "IW{1,2}(42,:)'" : Constant  Value=[-0.00795028964429910812994339863735149265266954898834228515625;0.006133615952391663177223346536948156426660716533660888671875;0.012792417644569280266164668091732892207801342010498046875;0.047536670714051799946364695870215655304491519927978515625;0.01857025425068357937785634703686810098588466644287109375]
      mask Display: e = 0.06;c1 = [120 150 230]/255;c2 = ([120 150 230]+0)/383;c3 = ([120 150 230]+128)/383;patch([0 1 1 0],[0 0 1 1],c1);patch([0 1 1 1-e 1-e 0+e],[0 0 1 1-e 0+e 0+e],c2);patch([0 0 1 1-e 0+e 0+e],[0 1 1 1-e 1-e 0+e],c3);plot([0 1 1 0 0],[0 0 1 1 0]);disp('Weights');
  "IW{1,2}(43,:)'" : Constant  Value=[0.00081676808839141966898933500118573647341690957546234130859375;0.0176598623328837640855670798600840498693287372589111328125;0.003015711371351383583705452195999896503053605556488037109375;0.05150230712044646941283332353123114444315433502197265625;0.0369312001607482176535057760702329687774181365966796875]
      mask Display: e = 0.06;c1 = [120 150 230]/255;c2 = ([120 150 230]+0)/383;c3 = ([120 150 230]+128)/383;patch([0 1 1 0],[0 0 1 1],c1);patch([0 1 1 1-e 1-e 0+e],[0 0 1 1-e 0+e 0+e],c2);patch([0 0 1 1-e 0+e 0+e],[0 1 1 1-e 1-e 0+e],c3);plot([0 1 1 0 0],[0 0 1 1 0]);disp('Weights');
  "IW{1,2}(44,:)'" : Constant  Value=[-0.12428194213717647098604857092141173779964447021484375;0.00666044380671207240929287962671878631226718425750732421875;0.0869411568591319794396810038961120881140232086181640625;0.09750588358359453533541483238877844996750354766845703125;-0.03342114122334023662563851075901766307651996612548828125]
      mask Display: e = 0.06;c1 = [120 150 230]/255;c2 = ([120 150 230]+0)/383;c3 = ([120 150 230]+128)/383;patch([0 1 1 0],[0 0 1 1],c1);patch([0 1 1 1-e 1-e 0+e],[0 0 1 1-e 0+e 0+e],c2);patch([0 0 1 1-e 0+e 0+e],[0 1 1 1-e 1-e 0+e],c3);plot([0 1 1 0 0],[0 0 1 1 0]);disp('Weights');
  "IW{1,2}(45,:)'" : Constant  Value=[-0.070816902067406040099939446008647792041301727294921875;0.0164454592017466948161708018005811027251183986663818359375;0.0120979832175336469990423182707672822289168834686279296875;-0.01165481095194141614168614751179120503365993499755859375;-0.006144824907584577056152141949496581219136714935302734375]
      mask Display: e = 0.06;c1 = [120 150 230]/255;c2 = ([120 150 230]+0)/383;c3 = ([120 150 230]+128)/383;patch([0 1 1 0],[0 0 1 1],c1);patch([0 1 1 1-e 1-e 0+e],[0 0 1 1-e 0+e 0+e],c2);patch([0 0 1 1-e 0+e 0+e],[0 1 1 1-e 1-e 0+e],c3);plot([0 1 1 0 0],[0 0 1 1 0]);disp('Weights');
  "IW{1,2}(46,:)'" : Constant  Value=[0.06534094260801122378001792867507901974022388458251953125;-0.0020051330823790364070446923250301551888696849346160888671875;-0.0691351110661047874028639625976211391389369964599609375;0.03938314660646664855381260395006393082439899444580078125;0.1470269811137322746308342402699054218828678131103515625]
      mask Display: e = 0.06;c1 = [120 150 230]/255;c2 = ([120 150 230]+0)/383;c3 = ([120 150 230]+128)/383;patch([0 1 1 0],[0 0 1 1],c1);patch([0 1 1 1-e 1-e 0+e],[0 0 1 1-e 0+e 0+e],c2);patch([0 0 1 1-e 0+e 0+e],[0 1 1 1-e 1-e 0+e],c3);plot([0 1 1 0 0],[0 0 1 1 0]);disp('Weights');
  "IW{1,2}(47,:)'" : Constant  Value=[0.053414398029033451076319494177369051612913608551025390625;-0.0070995937190487558299256676264121779240667819976806640625;0.005288393598413622213871843058541344362311065196990966796875;-0.04910093887565174231024656137378769926726818084716796875;-0.07764435610082069671999960291941533796489238739013671875]
      mask Display: e = 0.06;c1 = [120 150 230]/255;c2 = ([120 150 230]+0)/383;c3 = ([120 150 230]+128)/383;patch([0 1 1 0],[0 0 1 1],c1);patch([0 1 1 1-e 1-e 0+e],[0 0 1 1-e 0+e 0+e],c2);patch([0 0 1 1-e 0+e 0+e],[0 1 1 1-e 1-e 0+e],c3);plot([0 1 1 0 0],[0 0 1 1 0]);disp('Weights');
  "IW{1,2}(48,:)'" : Constant  Value=[-0.0702776772905580049410900755901820957660675048828125;-0.09318722565650006117721204645931720733642578125;0.10187113375325777819835337822951260022819042205810546875;0.107571740968418427808472870310652069747447967529296875;-0.06856554794930551366416437986117671243846416473388671875]
      mask Display: e = 0.06;c1 = [120 150 230]/255;c2 = ([120 150 230]+0)/383;c3 = ([120 150 230]+128)/383;patch([0 1 1 0],[0 0 1 1],c1);patch([0 1 1 1-e 1-e 0+e],[0 0 1 1-e 0+e 0+e],c2);patch([0 0 1 1-e 0+e 0+e],[0 1 1 1-e 1-e 0+e],c3);plot([0 1 1 0 0],[0 0 1 1 0]);disp('Weights');
  "IW{1,2}(49,:)'" : Constant  Value=[-0.0789589526203171576668182751745916903018951416015625;0.0092160245207722028826236027043705689720809459686279296875;0.03332445149348568780300894331958261318504810333251953125;-0.05270797359515333457835595254437066614627838134765625;-0.0815218709533274410450331970423576422035694122314453125]
      mask Display: e = 0.06;c1 = [120 150 230]/255;c2 = ([120 150 230]+0)/383;c3 = ([120 150 230]+128)/383;patch([0 1 1 0],[0 0 1 1],c1);patch([0 1 1 1-e 1-e 0+e],[0 0 1 1-e 0+e 0+e],c2);patch([0 0 1 1-e 0+e 0+e],[0 1 1 1-e 1-e 0+e],c3);plot([0 1 1 0 0],[0 0 1 1 0]);disp('Weights');
  "IW{1,2}(5,:)'" : Constant  Value=[0.010101402217861328580728041970360209234058856964111328125;-0.000614053077992773844138996164332411353825591504573822021484375;0.0195818187383685581026693256490034400485455989837646484375;0.01345489336628006259155565516039132489822804927825927734375;-0.0314055408235604238686988765039131976664066314697265625]
      mask Display: e = 0.06;c1 = [120 150 230]/255;c2 = ([120 150 230]+0)/383;c3 = ([120 150 230]+128)/383;patch([0 1 1 0],[0 0 1 1],c1);patch([0 1 1 1-e 1-e 0+e],[0 0 1 1-e 0+e 0+e],c2);patch([0 0 1 1-e 0+e 0+e],[0 1 1 1-e 1-e 0+e],c3);plot([0 1 1 0 0],[0 0 1 1 0]);disp('Weights');
  "IW{1,2}(50,:)'" : Constant  Value=[-0.19657692983947594456139995600096881389617919921875;0.0292269774182451237687363487793845706619322299957275390625;0.09124215886902618810605503085753298364579677581787109375;0.0166041726280283623295996875413038651458919048309326171875;-0.0846009140168149931238161798319197259843349456787109375]
      mask Display: e = 0.06;c1 = [120 150 230]/255;c2 = ([120 150 230]+0)/383;c3 = ([120 150 230]+128)/383;patch([0 1 1 0],[0 0 1 1],c1);patch([0 1 1 1-e 1-e 0+e],[0 0 1 1-e 0+e 0+e],c2);patch([0 0 1 1-e 0+e 0+e],[0 1 1 1-e 1-e 0+e],c3);plot([0 1 1 0 0],[0 0 1 1 0]);disp('Weights');
  "IW{1,2}(51,:)'" : Constant  Value=[-0.0200553937723044438390385124648673809133470058441162109375;0.005629485509033696315206451998847114737145602703094482421875;0.02691653991382693400513659298667334951460361480712890625;0.032985122986870930861247330767582752741873264312744140625;-0.0175287051223987945525184528605677769519388675689697265625]
      mask Display: e = 0.06;c1 = [120 150 230]/255;c2 = ([120 150 230]+0)/383;c3 = ([120 150 230]+128)/383;patch([0 1 1 0],[0 0 1 1],c1);patch([0 1 1 1-e 1-e 0+e],[0 0 1 1-e 0+e 0+e],c2);patch([0 0 1 1-e 0+e 0+e],[0 1 1 1-e 1-e 0+e],c3);plot([0 1 1 0 0],[0 0 1 1 0]);disp('Weights');
  "IW{1,2}(52,:)'" : Constant  Value=[0.0062086155728596041647460168633188004605472087860107421875;0.00514499081138465770568490853520415839739143848419189453125;0.01282012660580350051076070627686931402422487735748291015625;0.035715536835848125940540143119505955837666988372802734375;0.0028511173621683229099932344041690157609991729259490966796875]
      mask Display: e = 0.06;c1 = [120 150 230]/255;c2 = ([120 150 230]+0)/383;c3 = ([120 150 230]+128)/383;patch([0 1 1 0],[0 0 1 1],c1);patch([0 1 1 1-e 1-e 0+e],[0 0 1 1-e 0+e 0+e],c2);patch([0 0 1 1-e 0+e 0+e],[0 1 1 1-e 1-e 0+e],c3);plot([0 1 1 0 0],[0 0 1 1 0]);disp('Weights');
  "IW{1,2}(53,:)'" : Constant  Value=[0.035625044602090281953277184356920770369470119476318359375;0.009911032735840590024434249016849207691848278045654296875;0.0034697523988826846873256837255894424743019044399261474609375;-0.1373774560376276043793808412374346517026424407958984375;-0.155400431110711334525831261998973786830902099609375]
      mask Display: e = 0.06;c1 = [120 150 230]/255;c2 = ([120 150 230]+0)/383;c3 = ([120 150 230]+128)/383;patch([0 1 1 0],[0 0 1 1],c1);patch([0 1 1 1-e 1-e 0+e],[0 0 1 1-e 0+e 0+e],c2);patch([0 0 1 1-e 0+e 0+e],[0 1 1 1-e 1-e 0+e],c3);plot([0 1 1 0 0],[0 0 1 1 0]);disp('Weights');
  "IW{1,2}(54,:)'" : Constant  Value=[0.0195708586432779829689110329127288423478603363037109375;-0.00785360451670600971663116496301881852559745311737060546875;-0.045976299232901592095590359576817718334496021270751953125;0.0776790687028838799932373149204067885875701904296875;0.157043214364119332326907851893338374793529510498046875]
      mask Display: e = 0.06;c1 = [120 150 230]/255;c2 = ([120 150 230]+0)/383;c3 = ([120 150 230]+128)/383;patch([0 1 1 0],[0 0 1 1],c1);patch([0 1 1 1-e 1-e 0+e],[0 0 1 1-e 0+e 0+e],c2);patch([0 0 1 1-e 0+e 0+e],[0 1 1 1-e 1-e 0+e],c3);plot([0 1 1 0 0],[0 0 1 1 0]);disp('Weights');
  "IW{1,2}(55,:)'" : Constant  Value=[-0.04373920496144718950137786350751412101089954376220703125;0.0088617687558829767724422055152899702079594135284423828125;0.038734451467240797739588487047512899152934551239013671875;0.0663554185015422237636784075220930390059947967529296875;0.00026344708582784850427194189848023597733117640018463134765625]
      mask Display: e = 0.06;c1 = [120 150 230]/255;c2 = ([120 150 230]+0)/383;c3 = ([120 150 230]+128)/383;patch([0 1 1 0],[0 0 1 1],c1);patch([0 1 1 1-e 1-e 0+e],[0 0 1 1-e 0+e 0+e],c2);patch([0 0 1 1-e 0+e 0+e],[0 1 1 1-e 1-e 0+e],c3);plot([0 1 1 0 0],[0 0 1 1 0]);disp('Weights');
  "IW{1,2}(56,:)'" : Constant  Value=[0.029439535675457283170342037692535086534917354583740234375;0.0330578122322633394247759497375227510929107666015625;-0.019233955865888517633432996944975457154214382171630859375;0.049831584308810399075451158523719641380012035369873046875;0.0668206737120435045884647706770920194685459136962890625]
      mask Display: e = 0.06;c1 = [120 150 230]/255;c2 = ([120 150 230]+0)/383;c3 = ([120 150 230]+128)/383;patch([0 1 1 0],[0 0 1 1],c1);patch([0 1 1 1-e 1-e 0+e],[0 0 1 1-e 0+e 0+e],c2);patch([0 0 1 1-e 0+e 0+e],[0 1 1 1-e 1-e 0+e],c3);plot([0 1 1 0 0],[0 0 1 1 0]);disp('Weights');
  "IW{1,2}(57,:)'" : Constant  Value=[0.297532418440825840999508500317460857331752777099609375;-0.034088092708690620469269560999237000942230224609375;-0.14892102986354138760560772425378672778606414794921875;-0.0295061413700503753776427373622937011532485485076904296875;0.1429300612607231346640190849939244799315929412841796875]
      mask Display: e = 0.06;c1 = [120 150 230]/255;c2 = ([120 150 230]+0)/383;c3 = ([120 150 230]+128)/383;patch([0 1 1 0],[0 0 1 1],c1);patch([0 1 1 1-e 1-e 0+e],[0 0 1 1-e 0+e 0+e],c2);patch([0 0 1 1-e 0+e 0+e],[0 1 1 1-e 1-e 0+e],c3);plot([0 1 1 0 0],[0 0 1 1 0]);disp('Weights');
  "IW{1,2}(58,:)'" : Constant  Value=[0.046050588079049416256882665265948162414133548736572265625;-0.004610178140486079732818236465163863613270223140716552734375;-0.005728020777426158505196696069106110371649265289306640625;0.0489876732144139681590644386233179830014705657958984375;0.03693442596369800323685694820596836507320404052734375]
      mask Display: e = 0.06;c1 = [120 150 230]/255;c2 = ([120 150 230]+0)/383;c3 = ([120 150 230]+128)/383;patch([0 1 1 0],[0 0 1 1],c1);patch([0 1 1 1-e 1-e 0+e],[0 0 1 1-e 0+e 0+e],c2);patch([0 0 1 1-e 0+e 0+e],[0 1 1 1-e 1-e 0+e],c3);plot([0 1 1 0 0],[0 0 1 1 0]);disp('Weights');
  "IW{1,2}(59,:)'" : Constant  Value=[0.103009398151029163415159928263165056705474853515625;-0.0121680562744036456501728338253087713383138179779052734375;-0.07828735455464851111795354654532275162637233734130859375;-0.05780213635912208325340344572396134026348590850830078125;0.062596398520664620068743033698410727083683013916015625]
      mask Display: e = 0.06;c1 = [120 150 230]/255;c2 = ([120 150 230]+0)/383;c3 = ([120 150 230]+128)/383;patch([0 1 1 0],[0 0 1 1],c1);patch([0 1 1 1-e 1-e 0+e],[0 0 1 1-e 0+e 0+e],c2);patch([0 0 1 1-e 0+e 0+e],[0 1 1 1-e 1-e 0+e],c3);plot([0 1 1 0 0],[0 0 1 1 0]);disp('Weights');
  "IW{1,2}(6,:)'" : Constant  Value=[-0.0311791890698206904108946702081084367819130420684814453125;0.016995459719213755478417482436270802281796932220458984375;0.03188624420348902532840185131135513074696063995361328125;0.060422817949356659450454998250279459170997142791748046875;0.0030955897049768075525444377404937768005765974521636962890625]
      mask Display: e = 0.06;c1 = [120 150 230]/255;c2 = ([120 150 230]+0)/383;c3 = ([120 150 230]+128)/383;patch([0 1 1 0],[0 0 1 1],c1);patch([0 1 1 1-e 1-e 0+e],[0 0 1 1-e 0+e 0+e],c2);patch([0 0 1 1-e 0+e 0+e],[0 1 1 1-e 1-e 0+e],c3);plot([0 1 1 0 0],[0 0 1 1 0]);disp('Weights');
  "IW{1,2}(60,:)'" : Constant  Value=[-0.053186640687095491919489376186902518384158611297607421875;0.011134950294196067910323932892424636520445346832275390625;0.00869066832351204909823394473278312943875789642333984375;-0.043615569086009491062139176165146636776626110076904296875;-0.035103731099999264941846632837041397579014301300048828125]
      mask Display: e = 0.06;c1 = [120 150 230]/255;c2 = ([120 150 230]+0)/383;c3 = ([120 150 230]+128)/383;patch([0 1 1 0],[0 0 1 1],c1);patch([0 1 1 1-e 1-e 0+e],[0 0 1 1-e 0+e 0+e],c2);patch([0 0 1 1-e 0+e 0+e],[0 1 1 1-e 1-e 0+e],c3);plot([0 1 1 0 0],[0 0 1 1 0]);disp('Weights');
  "IW{1,2}(61,:)'" : Constant  Value=[0.04383895007263693965882112024701200425624847412109375;-0.00417775384777785245560277616050370852462947368621826171875;-0.05562356096120750492683981747177313081920146942138671875;-0.01632167143483632953948614385808468796312808990478515625;0.07791084271427604901472108167581609450280666351318359375]
      mask Display: e = 0.06;c1 = [120 150 230]/255;c2 = ([120 150 230]+0)/383;c3 = ([120 150 230]+128)/383;patch([0 1 1 0],[0 0 1 1],c1);patch([0 1 1 1-e 1-e 0+e],[0 0 1 1-e 0+e 0+e],c2);patch([0 0 1 1-e 0+e 0+e],[0 1 1 1-e 1-e 0+e],c3);plot([0 1 1 0 0],[0 0 1 1 0]);disp('Weights');
  "IW{1,2}(62,:)'" : Constant  Value=[-0.01163205148010725518969987746231709024868905544281005859375;0.005786232476052026452162380110166850499808788299560546875;0.0302453572830208954058672787823525140993297100067138671875;0.022926763495360942546330562663570162840187549591064453125;-0.035530279260345874747795136272543459199368953704833984375]
      mask Display: e = 0.06;c1 = [120 150 230]/255;c2 = ([120 150 230]+0)/383;c3 = ([120 150 230]+128)/383;patch([0 1 1 0],[0 0 1 1],c1);patch([0 1 1 1-e 1-e 0+e],[0 0 1 1-e 0+e 0+e],c2);patch([0 0 1 1-e 0+e 0+e],[0 1 1 1-e 1-e 0+e],c3);plot([0 1 1 0 0],[0 0 1 1 0]);disp('Weights');
  "IW{1,2}(63,:)'" : Constant  Value=[0.03548355233459417334973551305665750987827777862548828125;0.010527872219217644655930854469261248596012592315673828125;-0.011956914718693513466352129626102396287024021148681640625;0.030182421685183889736858731112079112790524959564208984375;0.03336747753743972422224572937921038828790187835693359375]
      mask Display: e = 0.06;c1 = [120 150 230]/255;c2 = ([120 150 230]+0)/383;c3 = ([120 150 230]+128)/383;patch([0 1 1 0],[0 0 1 1],c1);patch([0 1 1 1-e 1-e 0+e],[0 0 1 1-e 0+e 0+e],c2);patch([0 0 1 1-e 0+e 0+e],[0 1 1 1-e 1-e 0+e],c3);plot([0 1 1 0 0],[0 0 1 1 0]);disp('Weights');
  "IW{1,2}(64,:)'" : Constant  Value=[0.056500688265350491878979966031693038530647754669189453125;-0.0096651946281269170146988045644320663996040821075439453125;-0.044878679492911043025227257885489962063729763031005859375;-0.0646623951386925688300522097051725722849369049072265625;0.0091006982208810573153900946863359422422945499420166015625]
      mask Display: e = 0.06;c1 = [120 150 230]/255;c2 = ([120 150 230]+0)/383;c3 = ([120 150 230]+128)/383;patch([0 1 1 0],[0 0 1 1],c1);patch([0 1 1 1-e 1-e 0+e],[0 0 1 1-e 0+e 0+e],c2);patch([0 0 1 1-e 0+e 0+e],[0 1 1 1-e 1-e 0+e],c3);plot([0 1 1 0 0],[0 0 1 1 0]);disp('Weights');
  "IW{1,2}(65,:)'" : Constant  Value=[0.01416907376275116682562416059454335481859743595123291015625;0.0028483949521762781144362808305459111579693853855133056640625;0.0308722162659755931801708328521272051148116588592529296875;-0.04724337387927927955910689661322976462543010711669921875;-0.10979134175569719988896366658082115463912487030029296875]
      mask Display: e = 0.06;c1 = [120 150 230]/255;c2 = ([120 150 230]+0)/383;c3 = ([120 150 230]+128)/383;patch([0 1 1 0],[0 0 1 1],c1);patch([0 1 1 1-e 1-e 0+e],[0 0 1 1-e 0+e 0+e],c2);patch([0 0 1 1-e 0+e 0+e],[0 1 1 1-e 1-e 0+e],c3);plot([0 1 1 0 0],[0 0 1 1 0]);disp('Weights');
  "IW{1,2}(66,:)'" : Constant  Value=[0.037478006113766525186914435607832274399697780609130859375;-0.0280962849206550062397536038361067767255008220672607421875;0.00728610926092497675210513108368104440160095691680908203125;0.062707864274675007010273475316353142261505126953125;0.02898778434853831187378858658121316693723201751708984375]
      mask Display: e = 0.06;c1 = [120 150 230]/255;c2 = ([120 150 230]+0)/383;c3 = ([120 150 230]+128)/383;patch([0 1 1 0],[0 0 1 1],c1);patch([0 1 1 1-e 1-e 0+e],[0 0 1 1-e 0+e 0+e],c2);patch([0 0 1 1-e 0+e 0+e],[0 1 1 1-e 1-e 0+e],c3);plot([0 1 1 0 0],[0 0 1 1 0]);disp('Weights');
  "IW{1,2}(67,:)'" : Constant  Value=[-0.00623989977413751985280132572597722173668444156646728515625;0.0059009639551497634901711109023381141014397144317626953125;0.0334060075036575476747913171493564732372760772705078125;-0.003173055203902507004354305308879702351987361907958984375;-0.0674116744791228017508188941064872778952121734619140625]
      mask Display: e = 0.06;c1 = [120 150 230]/255;c2 = ([120 150 230]+0)/383;c3 = ([120 150 230]+128)/383;patch([0 1 1 0],[0 0 1 1],c1);patch([0 1 1 1-e 1-e 0+e],[0 0 1 1-e 0+e 0+e],c2);patch([0 0 1 1-e 0+e 0+e],[0 1 1 1-e 1-e 0+e],c3);plot([0 1 1 0 0],[0 0 1 1 0]);disp('Weights');
  "IW{1,2}(68,:)'" : Constant  Value=[-0.1285611480379074966773345067849732004106044769287109375;0.016943883999349783342491804205565131269395351409912109375;0.0850319704032116707725919013682869262993335723876953125;0.1059187758975919935178211517268209718167781829833984375;-0.0207655887558300146500389615766835049726068973541259765625]
      mask Display: e = 0.06;c1 = [120 150 230]/255;c2 = ([120 150 230]+0)/383;c3 = ([120 150 230]+128)/383;patch([0 1 1 0],[0 0 1 1],c1);patch([0 1 1 1-e 1-e 0+e],[0 0 1 1-e 0+e 0+e],c2);patch([0 0 1 1-e 0+e 0+e],[0 1 1 1-e 1-e 0+e],c3);plot([0 1 1 0 0],[0 0 1 1 0]);disp('Weights');
  "IW{1,2}(69,:)'" : Constant  Value=[0.168830699282009166761753249375033192336559295654296875;0.0359064220121265431640011911440524272620677947998046875;-0.082979500299221464754140242803259752690792083740234375;0.024969373544354224458974300659974687732756137847900390625;0.11331437167191658887954730516867130063474178314208984375]
      mask Display: e = 0.06;c1 = [120 150 230]/255;c2 = ([120 150 230]+0)/383;c3 = ([120 150 230]+128)/383;patch([0 1 1 0],[0 0 1 1],c1);patch([0 1 1 1-e 1-e 0+e],[0 0 1 1-e 0+e 0+e],c2);patch([0 0 1 1-e 0+e 0+e],[0 1 1 1-e 1-e 0+e],c3);plot([0 1 1 0 0],[0 0 1 1 0]);disp('Weights');
  "IW{1,2}(7,:)'" : Constant  Value=[-0.006280376853883662402466825369629077613353729248046875;-0.006448412693169601299369997349231198313646018505096435546875;-0.0202966079096140901427691716207846184261143207550048828125;-0.06175054801947814364648792206935468129813671112060546875;-0.0118466026803576811310403371635402436368167400360107421875]
      mask Display: e = 0.06;c1 = [120 150 230]/255;c2 = ([120 150 230]+0)/383;c3 = ([120 150 230]+128)/383;patch([0 1 1 0],[0 0 1 1],c1);patch([0 1 1 1-e 1-e 0+e],[0 0 1 1-e 0+e 0+e],c2);patch([0 0 1 1-e 0+e 0+e],[0 1 1 1-e 1-e 0+e],c3);plot([0 1 1 0 0],[0 0 1 1 0]);disp('Weights');
  "IW{1,2}(70,:)'" : Constant  Value=[0.02709614692098034904876868722567451186478137969970703125;-0.00906562667680456922558729360162033117376267910003662109375;-0.0203103458889562528411065756017706007696688175201416015625;-0.0708029415983756627017697837800369597971439361572265625;-0.03293545988036851446256747522056684829294681549072265625]
      mask Display: e = 0.06;c1 = [120 150 230]/255;c2 = ([120 150 230]+0)/383;c3 = ([120 150 230]+128)/383;patch([0 1 1 0],[0 0 1 1],c1);patch([0 1 1 1-e 1-e 0+e],[0 0 1 1-e 0+e 0+e],c2);patch([0 0 1 1-e 0+e 0+e],[0 1 1 1-e 1-e 0+e],c3);plot([0 1 1 0 0],[0 0 1 1 0]);disp('Weights');
  "IW{1,2}(71,:)'" : Constant  Value=[-0.1272734264441099105713561812081024982035160064697265625;0.01044732934238230825929605316559900529682636260986328125;0.049855817292208594315727765433621243573725223541259765625;0.170428366146471221842517707045772112905979156494140625;0.11685818113976141618959303514202474616467952728271484375]
      mask Display: e = 0.06;c1 = [120 150 230]/255;c2 = ([120 150 230]+0)/383;c3 = ([120 150 230]+128)/383;patch([0 1 1 0],[0 0 1 1],c1);patch([0 1 1 1-e 1-e 0+e],[0 0 1 1-e 0+e 0+e],c2);patch([0 0 1 1-e 0+e 0+e],[0 1 1 1-e 1-e 0+e],c3);plot([0 1 1 0 0],[0 0 1 1 0]);disp('Weights');
  "IW{1,2}(72,:)'" : Constant  Value=[0.01484401515593502217382759766906019649468362331390380859375;0.03218399273867970922236025899110245518386363983154296875;-0.002979484916718726228435087932666647247970104217529296875;0.067947213431189645849173075475846417248249053955078125;0.058928439543882070450475652023669681511819362640380859375]
      mask Display: e = 0.06;c1 = [120 150 230]/255;c2 = ([120 150 230]+0)/383;c3 = ([120 150 230]+128)/383;patch([0 1 1 0],[0 0 1 1],c1);patch([0 1 1 1-e 1-e 0+e],[0 0 1 1-e 0+e 0+e],c2);patch([0 0 1 1-e 0+e 0+e],[0 1 1 1-e 1-e 0+e],c3);plot([0 1 1 0 0],[0 0 1 1 0]);disp('Weights');
  "IW{1,2}(73,:)'" : Constant  Value=[-0.00662354827651624213091796633534613647498190402984619140625;-0.03330948348265920511135362858112785033881664276123046875;-0.0031173124861200236963842957749193374183960258960723876953125;-0.077467741809885526382828402347513474524021148681640625;-0.060641361550719898032557608757997513748705387115478515625]
      mask Display: e = 0.06;c1 = [120 150 230]/255;c2 = ([120 150 230]+0)/383;c3 = ([120 150 230]+128)/383;patch([0 1 1 0],[0 0 1 1],c1);patch([0 1 1 1-e 1-e 0+e],[0 0 1 1-e 0+e 0+e],c2);patch([0 0 1 1-e 0+e 0+e],[0 1 1 1-e 1-e 0+e],c3);plot([0 1 1 0 0],[0 0 1 1 0]);disp('Weights');
  "IW{1,2}(74,:)'" : Constant  Value=[-0.0765226744550026871660719507417525164783000946044921875;-0.0629949108643587940559172011489863507449626922607421875;0.0269826229678792606225812278353259898722171783447265625;-0.07232021250449793825509914313443005084991455078125;-0.08774125893122229624676577941499999724328517913818359375]
      mask Display: e = 0.06;c1 = [120 150 230]/255;c2 = ([120 150 230]+0)/383;c3 = ([120 150 230]+128)/383;patch([0 1 1 0],[0 0 1 1],c1);patch([0 1 1 1-e 1-e 0+e],[0 0 1 1-e 0+e 0+e],c2);patch([0 0 1 1-e 0+e 0+e],[0 1 1 1-e 1-e 0+e],c3);plot([0 1 1 0 0],[0 0 1 1 0]);disp('Weights');
  "IW{1,2}(75,:)'" : Constant  Value=[-0.05002424034769416272272479773164377547800540924072265625;-0.012413810162381681834187219237719546072185039520263671875;0.0392216032563809380295793971527018584311008453369140625;0.07817232206270242900192357637934037484228610992431640625;0.013632157583722957772121020525446510873734951019287109375]
      mask Display: e = 0.06;c1 = [120 150 230]/255;c2 = ([120 150 230]+0)/383;c3 = ([120 150 230]+128)/383;patch([0 1 1 0],[0 0 1 1],c1);patch([0 1 1 1-e 1-e 0+e],[0 0 1 1-e 0+e 0+e],c2);patch([0 0 1 1-e 0+e 0+e],[0 1 1 1-e 1-e 0+e],c3);plot([0 1 1 0 0],[0 0 1 1 0]);disp('Weights');
  "IW{1,2}(76,:)'" : Constant  Value=[0.0298647443345664322100763143907897756434977054595947265625;-0.02763319342700609748675333321443758904933929443359375;-0.01544331563243443554422906771605994435958564281463623046875;-0.07936006184212930636423521946198889054358005523681640625;-0.05050877487341998151038069408969022333621978759765625]
      mask Display: e = 0.06;c1 = [120 150 230]/255;c2 = ([120 150 230]+0)/383;c3 = ([120 150 230]+128)/383;patch([0 1 1 0],[0 0 1 1],c1);patch([0 1 1 1-e 1-e 0+e],[0 0 1 1-e 0+e 0+e],c2);patch([0 0 1 1-e 0+e 0+e],[0 1 1 1-e 1-e 0+e],c3);plot([0 1 1 0 0],[0 0 1 1 0]);disp('Weights');
  "IW{1,2}(77,:)'" : Constant  Value=[-0.01169332349246907619411128820274825557135045528411865234375;0.1443364276033036464053083136604982428252696990966796875;-0.04952655687030636799672578263198374770581722259521484375;0.0249240366059819036526068458670124527998268604278564453125;0.11632002061284037186528195206847158260643482208251953125]
      mask Display: e = 0.06;c1 = [120 150 230]/255;c2 = ([120 150 230]+0)/383;c3 = ([120 150 230]+128)/383;patch([0 1 1 0],[0 0 1 1],c1);patch([0 1 1 1-e 1-e 0+e],[0 0 1 1-e 0+e 0+e],c2);patch([0 0 1 1-e 0+e 0+e],[0 1 1 1-e 1-e 0+e],c3);plot([0 1 1 0 0],[0 0 1 1 0]);disp('Weights');
  "IW{1,2}(78,:)'" : Constant  Value=[-0.0020125174748483166085877282824867506860755383968353271484375;0.03190546428362150965796217860770411789417266845703125;-0.004882234453004231401751500385444160201586782932281494140625;0.1497948535376275314145999573156586848199367523193359375;0.1596592009022403668705436530217411927878856658935546875]
      mask Display: e = 0.06;c1 = [120 150 230]/255;c2 = ([120 150 230]+0)/383;c3 = ([120 150 230]+128)/383;patch([0 1 1 0],[0 0 1 1],c1);patch([0 1 1 1-e 1-e 0+e],[0 0 1 1-e 0+e 0+e],c2);patch([0 0 1 1-e 0+e 0+e],[0 1 1 1-e 1-e 0+e],c3);plot([0 1 1 0 0],[0 0 1 1 0]);disp('Weights');
  "IW{1,2}(79,:)'" : Constant  Value=[-0.0228717565017696779217093450142783694900572299957275390625;0.001759787609959452374386312811793686705641448497772216796875;-0.0252986868881747810344773341739710303954780101776123046875;0.0307986727002874383085639919954701326787471771240234375;0.0863401148481389990596568395631038583815097808837890625]
      mask Display: e = 0.06;c1 = [120 150 230]/255;c2 = ([120 150 230]+0)/383;c3 = ([120 150 230]+128)/383;patch([0 1 1 0],[0 0 1 1],c1);patch([0 1 1 1-e 1-e 0+e],[0 0 1 1-e 0+e 0+e],c2);patch([0 0 1 1-e 0+e 0+e],[0 1 1 1-e 1-e 0+e],c3);plot([0 1 1 0 0],[0 0 1 1 0]);disp('Weights');
  "IW{1,2}(8,:)'" : Constant  Value=[0.046367108880403858084395807281907764263451099395751953125;0.00168542206739497242053149594909200459369458258152008056640625;0.01183222638417159335022521560176755883730947971343994140625;-0.0664061407782430002111340172632480971515178680419921875;-0.10325489235921285480213072105470928363502025604248046875]
      mask Display: e = 0.06;c1 = [120 150 230]/255;c2 = ([120 150 230]+0)/383;c3 = ([120 150 230]+128)/383;patch([0 1 1 0],[0 0 1 1],c1);patch([0 1 1 1-e 1-e 0+e],[0 0 1 1-e 0+e 0+e],c2);patch([0 0 1 1-e 0+e 0+e],[0 1 1 1-e 1-e 0+e],c3);plot([0 1 1 0 0],[0 0 1 1 0]);disp('Weights');
  "IW{1,2}(80,:)'" : Constant  Value=[0.00242433973091161526769443668172243633307516574859619140625;-0.0084130955172444059353420442448623361997306346893310546875;0.01336072432992155799291733586642294540069997310638427734375;0.063182555118927063997347204349352978169918060302734375;0.0307155057896809254025516366937154089100658893585205078125]
      mask Display: e = 0.06;c1 = [120 150 230]/255;c2 = ([120 150 230]+0)/383;c3 = ([120 150 230]+128)/383;patch([0 1 1 0],[0 0 1 1],c1);patch([0 1 1 1-e 1-e 0+e],[0 0 1 1-e 0+e 0+e],c2);patch([0 0 1 1-e 0+e 0+e],[0 1 1 1-e 1-e 0+e],c3);plot([0 1 1 0 0],[0 0 1 1 0]);disp('Weights');
  "IW{1,2}(81,:)'" : Constant  Value=[-0.041904425666155951935021306553608155809342861175537109375;0.00658958792671388536577037342567564337514340877532958984375;0.03552023322501186852750976186143816448748111724853515625;-0.1151146335386567243208588706693262793123722076416015625;-0.168513629193430436448153386663761921226978302001953125]
      mask Display: e = 0.06;c1 = [120 150 230]/255;c2 = ([120 150 230]+0)/383;c3 = ([120 150 230]+128)/383;patch([0 1 1 0],[0 0 1 1],c1);patch([0 1 1 1-e 1-e 0+e],[0 0 1 1-e 0+e 0+e],c2);patch([0 0 1 1-e 0+e 0+e],[0 1 1 1-e 1-e 0+e],c3);plot([0 1 1 0 0],[0 0 1 1 0]);disp('Weights');
  "IW{1,2}(82,:)'" : Constant  Value=[-0.00889638500304427808085261375481422874145209789276123046875;0.00324502319811211491218383429213645285926759243011474609375;-0.0311693975373349592417060449633936514146625995635986328125;0.0204825654171228201116949918514364981092512607574462890625;0.08338868488624584518476012817700393497943878173828125]
      mask Display: e = 0.06;c1 = [120 150 230]/255;c2 = ([120 150 230]+0)/383;c3 = ([120 150 230]+128)/383;patch([0 1 1 0],[0 0 1 1],c1);patch([0 1 1 1-e 1-e 0+e],[0 0 1 1-e 0+e 0+e],c2);patch([0 0 1 1-e 0+e 0+e],[0 1 1 1-e 1-e 0+e],c3);plot([0 1 1 0 0],[0 0 1 1 0]);disp('Weights');
  "IW{1,2}(83,:)'" : Constant  Value=[-0.01676547506257063113732641568276449106633663177490234375;0.0087035631759373177640526364484685473144054412841796875;-0.01056046042669889391263371436480156262405216693878173828125;-0.066715153697562257217867909275810234248638153076171875;-0.032808911994657748156800636252228287048637866973876953125]
      mask Display: e = 0.06;c1 = [120 150 230]/255;c2 = ([120 150 230]+0)/383;c3 = ([120 150 230]+128)/383;patch([0 1 1 0],[0 0 1 1],c1);patch([0 1 1 1-e 1-e 0+e],[0 0 1 1-e 0+e 0+e],c2);patch([0 0 1 1-e 0+e 0+e],[0 1 1 1-e 1-e 0+e],c3);plot([0 1 1 0 0],[0 0 1 1 0]);disp('Weights');
  "IW{1,2}(84,:)'" : Constant  Value=[0.0123130098307969275406303921727158012799918651580810546875;0.0028049269645423970283293346739128537592478096485137939453125;0.00824660145692025954577974999892830965109169483184814453125;0.0722092022054929838503767314250580966472625732421875;0.04357217270310827228474437333716196008026599884033203125]
      mask Display: e = 0.06;c1 = [120 150 230]/255;c2 = ([120 150 230]+0)/383;c3 = ([120 150 230]+128)/383;patch([0 1 1 0],[0 0 1 1],c1);patch([0 1 1 1-e 1-e 0+e],[0 0 1 1-e 0+e 0+e],c2);patch([0 0 1 1-e 0+e 0+e],[0 1 1 1-e 1-e 0+e],c3);plot([0 1 1 0 0],[0 0 1 1 0]);disp('Weights');
  "IW{1,2}(85,:)'" : Constant  Value=[-0.038722078893211213379554891389489057473838329315185546875;0.001744540471324718990120405948118786909617483615875244140625;-0.0172082590616888277124107986537637771107256412506103515625;0.036617758892380190827164909705970785580575466156005859375;0.0819038563665162033800015706219710409641265869140625]
      mask Display: e = 0.06;c1 = [120 150 230]/255;c2 = ([120 150 230]+0)/383;c3 = ([120 150 230]+128)/383;patch([0 1 1 0],[0 0 1 1],c1);patch([0 1 1 1-e 1-e 0+e],[0 0 1 1-e 0+e 0+e],c2);patch([0 0 1 1-e 0+e 0+e],[0 1 1 1-e 1-e 0+e],c3);plot([0 1 1 0 0],[0 0 1 1 0]);disp('Weights');
  "IW{1,2}(86,:)'" : Constant  Value=[0.047117637426651516607822856030907132662832736968994140625;-0.028827455596412303318043512945223483256995677947998046875;0.00550958456487406385282401544145614025183022022247314453125;-0.0512290298363665963510271694758557714521884918212890625;-0.07661456142018625847800450401337002404034137725830078125]
      mask Display: e = 0.06;c1 = [120 150 230]/255;c2 = ([120 150 230]+0)/383;c3 = ([120 150 230]+128)/383;patch([0 1 1 0],[0 0 1 1],c1);patch([0 1 1 1-e 1-e 0+e],[0 0 1 1-e 0+e 0+e],c2);patch([0 0 1 1-e 0+e 0+e],[0 1 1 1-e 1-e 0+e],c3);plot([0 1 1 0 0],[0 0 1 1 0]);disp('Weights');
  "IW{1,2}(87,:)'" : Constant  Value=[-0.0020655813471467938773062922308554334449581801891326904296875;0.00776598610027402248834338394090082147158682346343994140625;0.01439942258983055445309418018950964324176311492919921875;0.044821573730011103620096690747232059948146343231201171875;0.01110380335180936005323726334381717606447637081146240234375]
      mask Display: e = 0.06;c1 = [120 150 230]/255;c2 = ([120 150 230]+0)/383;c3 = ([120 150 230]+128)/383;patch([0 1 1 0],[0 0 1 1],c1);patch([0 1 1 1-e 1-e 0+e],[0 0 1 1-e 0+e 0+e],c2);patch([0 0 1 1-e 0+e 0+e],[0 1 1 1-e 1-e 0+e],c3);plot([0 1 1 0 0],[0 0 1 1 0]);disp('Weights');
  "IW{1,2}(88,:)'" : Constant  Value=[-0.0160733094294609468732915047439746558666229248046875;0.00090557772402789890771324099461025980417616665363311767578125;0.03446369187478293127924189320765435695648193359375;0.02109689649226643981538842353984364308416843414306640625;-0.043419023846199673866141921507733059115707874298095703125]
      mask Display: e = 0.06;c1 = [120 150 230]/255;c2 = ([120 150 230]+0)/383;c3 = ([120 150 230]+128)/383;patch([0 1 1 0],[0 0 1 1],c1);patch([0 1 1 1-e 1-e 0+e],[0 0 1 1-e 0+e 0+e],c2);patch([0 0 1 1-e 0+e 0+e],[0 1 1 1-e 1-e 0+e],c3);plot([0 1 1 0 0],[0 0 1 1 0]);disp('Weights');
  "IW{1,2}(89,:)'" : Constant  Value=[-0.03500763577537240045511879316109116189181804656982421875;-0.001634813641418610651034892811139798141084611415863037109375;-0.018839114131199700963303911294133285991847515106201171875;0.08585685954516643347833593225004733540117740631103515625;0.131350736620477082094993193095433525741100311279296875]
      mask Display: e = 0.06;c1 = [120 150 230]/255;c2 = ([120 150 230]+0)/383;c3 = ([120 150 230]+128)/383;patch([0 1 1 0],[0 0 1 1],c1);patch([0 1 1 1-e 1-e 0+e],[0 0 1 1-e 0+e 0+e],c2);patch([0 0 1 1-e 0+e 0+e],[0 1 1 1-e 1-e 0+e],c3);plot([0 1 1 0 0],[0 0 1 1 0]);disp('Weights');
  "IW{1,2}(9,:)'" : Constant  Value=[-0.0484976420463635593538498369525768794119358062744140625;-0.00339367449206574335607289327754187979735434055328369140625;0.01252502066403327236898679331034145434387028217315673828125;-0.052184635040541549333426019074977375566959381103515625;-0.051245774833881395371459888110621250234544277191162109375]
      mask Display: e = 0.06;c1 = [120 150 230]/255;c2 = ([120 150 230]+0)/383;c3 = ([120 150 230]+128)/383;patch([0 1 1 0],[0 0 1 1],c1);patch([0 1 1 1-e 1-e 0+e],[0 0 1 1-e 0+e 0+e],c2);patch([0 0 1 1-e 0+e 0+e],[0 1 1 1-e 1-e 0+e],c3);plot([0 1 1 0 0],[0 0 1 1 0]);disp('Weights');
  "IW{1,2}(90,:)'" : Constant  Value=[-0.0109176261920139218430936267623110325075685977935791015625;0.0288048532074580802830876535836068796925246715545654296875;0.00981009956273464801823624981125249178148806095123291015625;0.073950472324662841483444708501338027417659759521484375;0.050421857216715236515991449550710967741906642913818359375]
      mask Display: e = 0.06;c1 = [120 150 230]/255;c2 = ([120 150 230]+0)/383;c3 = ([120 150 230]+128)/383;patch([0 1 1 0],[0 0 1 1],c1);patch([0 1 1 1-e 1-e 0+e],[0 0 1 1-e 0+e 0+e],c2);patch([0 0 1 1-e 0+e 0+e],[0 1 1 1-e 1-e 0+e],c3);plot([0 1 1 0 0],[0 0 1 1 0]);disp('Weights');
  "IW{1,2}(91,:)'" : Constant  Value=[-0.07827795306876676739715747999071027152240276336669921875;-0.007125604461579477556798511983515709289349615573883056640625;0.044951549018300514248824839569351752288639545440673828125;-0.087301579693083664057695614246767945587635040283203125;-0.145779803851686262650133585339062847197055816650390625]
      mask Display: e = 0.06;c1 = [120 150 230]/255;c2 = ([120 150 230]+0)/383;c3 = ([120 150 230]+128)/383;patch([0 1 1 0],[0 0 1 1],c1);patch([0 1 1 1-e 1-e 0+e],[0 0 1 1-e 0+e 0+e],c2);patch([0 0 1 1-e 0+e 0+e],[0 1 1 1-e 1-e 0+e],c3);plot([0 1 1 0 0],[0 0 1 1 0]);disp('Weights');
  "IW{1,2}(92,:)'" : Constant  Value=[-0.0233443560700996068091317425796660245396196842193603515625;-0.01965661959004581793575283654718077741563320159912109375;0.038956501539266837064179327398960595019161701202392578125;0.0666932513252659064928451471132575534284114837646484375;-0.00443994214356853607317265897336255875416100025177001953125]
      mask Display: e = 0.06;c1 = [120 150 230]/255;c2 = ([120 150 230]+0)/383;c3 = ([120 150 230]+128)/383;patch([0 1 1 0],[0 0 1 1],c1);patch([0 1 1 1-e 1-e 0+e],[0 0 1 1-e 0+e 0+e],c2);patch([0 0 1 1-e 0+e 0+e],[0 1 1 1-e 1-e 0+e],c3);plot([0 1 1 0 0],[0 0 1 1 0]);disp('Weights');
  "IW{1,2}(93,:)'" : Constant  Value=[-0.0280614865884632226633588203412728034891188144683837890625;0.0101067236352357751882902192619440029375255107879638671875;0.040459119539689593347819851487656706012785434722900390625;0.019032632102801587403728689196213963441550731658935546875;-0.05312932529971307882288300561413052491843700408935546875]
      mask Display: e = 0.06;c1 = [120 150 230]/255;c2 = ([120 150 230]+0)/383;c3 = ([120 150 230]+128)/383;patch([0 1 1 0],[0 0 1 1],c1);patch([0 1 1 1-e 1-e 0+e],[0 0 1 1-e 0+e 0+e],c2);patch([0 0 1 1-e 0+e 0+e],[0 1 1 1-e 1-e 0+e],c3);plot([0 1 1 0 0],[0 0 1 1 0]);disp('Weights');
  "IW{1,2}(94,:)'" : Constant  Value=[-0.0180237435453893431180905082555909757502377033233642578125;-0.00149831599683425431036865038691985319019295275211334228515625;-0.005911199091877290291707769398499294766224920749664306640625;-0.023213413815095083891915095364311127923429012298583984375;-0.0033078482348178768999991117283343555754981935024261474609375]
      mask Display: e = 0.06;c1 = [120 150 230]/255;c2 = ([120 150 230]+0)/383;c3 = ([120 150 230]+128)/383;patch([0 1 1 0],[0 0 1 1],c1);patch([0 1 1 1-e 1-e 0+e],[0 0 1 1-e 0+e 0+e],c2);patch([0 0 1 1-e 0+e 0+e],[0 1 1 1-e 1-e 0+e],c3);plot([0 1 1 0 0],[0 0 1 1 0]);disp('Weights');
  "IW{1,2}(95,:)'" : Constant  Value=[-0.1298459062237030947617455467479885555803775787353515625;0.05535958711240472618353436473626061342656612396240234375;0.054034599075738924678358188202764722518622875213623046875;0.164507728636724748216835223502130247652530670166015625;0.10315145429831747148075038467140984721481800079345703125]
      mask Display: e = 0.06;c1 = [120 150 230]/255;c2 = ([120 150 230]+0)/383;c3 = ([120 150 230]+128)/383;patch([0 1 1 0],[0 0 1 1],c1);patch([0 1 1 1-e 1-e 0+e],[0 0 1 1-e 0+e 0+e],c2);patch([0 0 1 1-e 0+e 0+e],[0 1 1 1-e 1-e 0+e],c3);plot([0 1 1 0 0],[0 0 1 1 0]);disp('Weights');
  "IW{1,2}(96,:)'" : Constant  Value=[-0.002908889833235703097080726564627184416167438030242919921875;0.044609472269952023248951178402421646751463413238525390625;0.00999226594835701809049766097814426757395267486572265625;0.1342387674244666373457590680118300952017307281494140625;0.10872887514901850847248709897030494175851345062255859375]
      mask Display: e = 0.06;c1 = [120 150 230]/255;c2 = ([120 150 230]+0)/383;c3 = ([120 150 230]+128)/383;patch([0 1 1 0],[0 0 1 1],c1);patch([0 1 1 1-e 1-e 0+e],[0 0 1 1-e 0+e 0+e],c2);patch([0 0 1 1-e 0+e 0+e],[0 1 1 1-e 1-e 0+e],c3);plot([0 1 1 0 0],[0 0 1 1 0]);disp('Weights');
  "IW{1,2}(97,:)'" : Constant  Value=[-0.030185176680019236428176299114056746475398540496826171875;-0.0021777377495732544963880084054608232690952718257904052734375;-0.0017585751410032321624676843185852703754790127277374267578125;-0.0137349325040490473359700018818330136127769947052001953125;0.005187639615479648115548005904429373913444578647613525390625]
      mask Display: e = 0.06;c1 = [120 150 230]/255;c2 = ([120 150 230]+0)/383;c3 = ([120 150 230]+128)/383;patch([0 1 1 0],[0 0 1 1],c1);patch([0 1 1 1-e 1-e 0+e],[0 0 1 1-e 0+e 0+e],c2);patch([0 0 1 1-e 0+e 0+e],[0 1 1 1-e 1-e 0+e],c3);plot([0 1 1 0 0],[0 0 1 1 0]);disp('Weights');
  "IW{1,2}(98,:)'" : Constant  Value=[-0.054757069687668080693043748397030867636203765869140625;0.015329329474747556416591720562792033888399600982666015625;0.047266643743484597350867915110939065925776958465576171875;0.0415885492312116078483796854925458319485187530517578125;-0.036417128879369480010108617307196254841983318328857421875]
      mask Display: e = 0.06;c1 = [120 150 230]/255;c2 = ([120 150 230]+0)/383;c3 = ([120 150 230]+128)/383;patch([0 1 1 0],[0 0 1 1],c1);patch([0 1 1 1-e 1-e 0+e],[0 0 1 1-e 0+e 0+e],c2);patch([0 0 1 1-e 0+e 0+e],[0 1 1 1-e 1-e 0+e],c3);plot([0 1 1 0 0],[0 0 1 1 0]);disp('Weights');
  "IW{1,2}(99,:)'" : Constant  Value=[0.041943843354097794240420427058779750950634479522705078125;0.046909351896642102752732483850195421837270259857177734375;-0.021381639625762616230275625639478676021099090576171875;0.045995326965924621109849113054224289953708648681640625;0.06251407402016632974817156309654819779098033905029296875]
      mask Display: e = 0.06;c1 = [120 150 230]/255;c2 = ([120 150 230]+0)/383;c3 = ([120 150 230]+128)/383;patch([0 1 1 0],[0 0 1 1],c1);patch([0 1 1 1-e 1-e 0+e],[0 0 1 1-e 0+e 0+e],c2);patch([0 0 1 1-e 0+e 0+e],[0 1 1 1-e 1-e 0+e],c3);plot([0 1 1 0 0],[0 0 1 1 0]);disp('Weights');
  Mux : Mux  Inputs=125
      mask Display: e = 0.06;c1 = [120 150 230]/255;c2 = ([120 150 230]+0)/383;c3 = ([120 150 230]+128)/383;patch([0 1 1 0],[0 0 1 1],c1);patch([0 1 1 1-e 1-e 0+e],[0 0 1 1-e 0+e 0+e],c2);patch([0 0 1 1-e 0+e 0+e],[0 1 1 1-e 1-e 0+e],c3);plot([0 1 1 0 0],[0 0 1 1 0]);disp('Mux');
  dotprod{1..125} (125 alike) : neural/Weight Functions/dotprod
  "iz{1,2}" : Outport
      mask Display: e = 0.06;c1 = [120 230 180]/255;c2 = ([120 230 180]+0)/(256+128);c3 = ([120 230 180]+128)/(256+128);patch([0 1 1 0],[0 0 1 1],c1);patch([0 1 1 1-e 1-e 0+e],[0 0 1 1-e 0+e 0+e],c2);patch([0 0 1 1-e 0+e 0+e],[0 1 1 1-e 1-e 0+e],c3);plot([0 1 1 0 0],[0 0 1 1 0]);
  wires:
  Mux/1 -> "iz{1,2}"/1
  dotprod125/1 -> Mux/125
  "IW{1,2}(125,:)'"/1 -> dotprod125/1
  dotprod124/1 -> Mux/124
  "IW{1,2}(124,:)'"/1 -> dotprod124/1
  dotprod123/1 -> Mux/123
  "IW{1,2}(123,:)'"/1 -> dotprod123/1
  dotprod122/1 -> Mux/122
  "IW{1,2}(122,:)'"/1 -> dotprod122/1
  dotprod121/1 -> Mux/121
  "IW{1,2}(121,:)'"/1 -> dotprod121/1
  dotprod120/1 -> Mux/120
  "IW{1,2}(120,:)'"/1 -> dotprod120/1
  dotprod119/1 -> Mux/119
  "IW{1,2}(119,:)'"/1 -> dotprod119/1
  dotprod118/1 -> Mux/118
  "IW{1,2}(118,:)'"/1 -> dotprod118/1
  dotprod117/1 -> Mux/117
  "IW{1,2}(117,:)'"/1 -> dotprod117/1
  dotprod116/1 -> Mux/116
  "IW{1,2}(116,:)'"/1 -> dotprod116/1
  dotprod115/1 -> Mux/115
  "IW{1,2}(115,:)'"/1 -> dotprod115/1
  dotprod114/1 -> Mux/114
  "IW{1,2}(114,:)'"/1 -> dotprod114/1
  dotprod113/1 -> Mux/113
  "IW{1,2}(113,:)'"/1 -> dotprod113/1
  dotprod112/1 -> Mux/112
  "IW{1,2}(112,:)'"/1 -> dotprod112/1
  dotprod111/1 -> Mux/111
  "IW{1,2}(111,:)'"/1 -> dotprod111/1
  dotprod110/1 -> Mux/110
  "IW{1,2}(110,:)'"/1 -> dotprod110/1
  dotprod109/1 -> Mux/109
  "IW{1,2}(109,:)'"/1 -> dotprod109/1
  dotprod108/1 -> Mux/108
  "IW{1,2}(108,:)'"/1 -> dotprod108/1
  dotprod107/1 -> Mux/107
  "IW{1,2}(107,:)'"/1 -> dotprod107/1
  dotprod106/1 -> Mux/106
  "IW{1,2}(106,:)'"/1 -> dotprod106/1
  dotprod105/1 -> Mux/105
  "IW{1,2}(105,:)'"/1 -> dotprod105/1
  dotprod104/1 -> Mux/104
  "IW{1,2}(104,:)'"/1 -> dotprod104/1
  dotprod103/1 -> Mux/103
  "IW{1,2}(103,:)'"/1 -> dotprod103/1
  dotprod102/1 -> Mux/102
  "IW{1,2}(102,:)'"/1 -> dotprod102/1
  dotprod101/1 -> Mux/101
  "IW{1,2}(101,:)'"/1 -> dotprod101/1
  dotprod100/1 -> Mux/100
  "IW{1,2}(100,:)'"/1 -> dotprod100/1
  dotprod99/1 -> Mux/99
  "IW{1,2}(99,:)'"/1 -> dotprod99/1
  dotprod98/1 -> Mux/98
  "IW{1,2}(98,:)'"/1 -> dotprod98/1
  dotprod97/1 -> Mux/97
  "IW{1,2}(97,:)'"/1 -> dotprod97/1
  dotprod96/1 -> Mux/96
  "IW{1,2}(96,:)'"/1 -> dotprod96/1
  dotprod95/1 -> Mux/95
  "IW{1,2}(95,:)'"/1 -> dotprod95/1
  dotprod94/1 -> Mux/94
  "IW{1,2}(94,:)'"/1 -> dotprod94/1
  dotprod93/1 -> Mux/93
  "IW{1,2}(93,:)'"/1 -> dotprod93/1
  dotprod92/1 -> Mux/92
  "IW{1,2}(92,:)'"/1 -> dotprod92/1
  dotprod91/1 -> Mux/91
  "IW{1,2}(91,:)'"/1 -> dotprod91/1
  dotprod90/1 -> Mux/90
  "IW{1,2}(90,:)'"/1 -> dotprod90/1
  dotprod89/1 -> Mux/89
  "IW{1,2}(89,:)'"/1 -> dotprod89/1
  dotprod88/1 -> Mux/88
  "IW{1,2}(88,:)'"/1 -> dotprod88/1
  dotprod87/1 -> Mux/87
  "IW{1,2}(87,:)'"/1 -> dotprod87/1
  dotprod86/1 -> Mux/86
  "IW{1,2}(86,:)'"/1 -> dotprod86/1
  dotprod85/1 -> Mux/85
  "IW{1,2}(85,:)'"/1 -> dotprod85/1
  dotprod84/1 -> Mux/84
  "IW{1,2}(84,:)'"/1 -> dotprod84/1
  dotprod83/1 -> Mux/83
  "IW{1,2}(83,:)'"/1 -> dotprod83/1
  dotprod82/1 -> Mux/82
  "IW{1,2}(82,:)'"/1 -> dotprod82/1
  dotprod81/1 -> Mux/81
  "IW{1,2}(81,:)'"/1 -> dotprod81/1
  dotprod80/1 -> Mux/80
  "IW{1,2}(80,:)'"/1 -> dotprod80/1
  dotprod79/1 -> Mux/79
  "IW{1,2}(79,:)'"/1 -> dotprod79/1
  dotprod78/1 -> Mux/78
  "IW{1,2}(78,:)'"/1 -> dotprod78/1
  dotprod77/1 -> Mux/77
  "IW{1,2}(77,:)'"/1 -> dotprod77/1
  dotprod76/1 -> Mux/76
  "IW{1,2}(76,:)'"/1 -> dotprod76/1
  dotprod75/1 -> Mux/75
  "IW{1,2}(75,:)'"/1 -> dotprod75/1
  dotprod74/1 -> Mux/74
  "IW{1,2}(74,:)'"/1 -> dotprod74/1
  dotprod73/1 -> Mux/73
  "IW{1,2}(73,:)'"/1 -> dotprod73/1
  dotprod72/1 -> Mux/72
  "IW{1,2}(72,:)'"/1 -> dotprod72/1
  dotprod71/1 -> Mux/71
  "IW{1,2}(71,:)'"/1 -> dotprod71/1
  dotprod70/1 -> Mux/70
  "IW{1,2}(70,:)'"/1 -> dotprod70/1
  dotprod69/1 -> Mux/69
  "IW{1,2}(69,:)'"/1 -> dotprod69/1
  dotprod68/1 -> Mux/68
  "IW{1,2}(68,:)'"/1 -> dotprod68/1
  dotprod67/1 -> Mux/67
  "IW{1,2}(67,:)'"/1 -> dotprod67/1
  dotprod66/1 -> Mux/66
  "IW{1,2}(66,:)'"/1 -> dotprod66/1
  dotprod65/1 -> Mux/65
  "IW{1,2}(65,:)'"/1 -> dotprod65/1
  dotprod64/1 -> Mux/64
  "IW{1,2}(64,:)'"/1 -> dotprod64/1
  dotprod63/1 -> Mux/63
  "IW{1,2}(63,:)'"/1 -> dotprod63/1
  dotprod62/1 -> Mux/62
  "IW{1,2}(62,:)'"/1 -> dotprod62/1
  dotprod61/1 -> Mux/61
  "IW{1,2}(61,:)'"/1 -> dotprod61/1
  dotprod60/1 -> Mux/60
  "IW{1,2}(60,:)'"/1 -> dotprod60/1
  dotprod59/1 -> Mux/59
  "IW{1,2}(59,:)'"/1 -> dotprod59/1
  dotprod58/1 -> Mux/58
  "IW{1,2}(58,:)'"/1 -> dotprod58/1
  dotprod57/1 -> Mux/57
  "IW{1,2}(57,:)'"/1 -> dotprod57/1
  dotprod56/1 -> Mux/56
  "IW{1,2}(56,:)'"/1 -> dotprod56/1
  dotprod55/1 -> Mux/55
  "IW{1,2}(55,:)'"/1 -> dotprod55/1
  dotprod54/1 -> Mux/54
  "IW{1,2}(54,:)'"/1 -> dotprod54/1
  dotprod53/1 -> Mux/53
  "IW{1,2}(53,:)'"/1 -> dotprod53/1
  dotprod52/1 -> Mux/52
  "IW{1,2}(52,:)'"/1 -> dotprod52/1
  dotprod51/1 -> Mux/51
  "IW{1,2}(51,:)'"/1 -> dotprod51/1
  dotprod50/1 -> Mux/50
  "IW{1,2}(50,:)'"/1 -> dotprod50/1
  dotprod49/1 -> Mux/49
  "IW{1,2}(49,:)'"/1 -> dotprod49/1
  dotprod48/1 -> Mux/48
  "IW{1,2}(48,:)'"/1 -> dotprod48/1
  dotprod47/1 -> Mux/47
  "IW{1,2}(47,:)'"/1 -> dotprod47/1
  dotprod46/1 -> Mux/46
  "IW{1,2}(46,:)'"/1 -> dotprod46/1
  dotprod45/1 -> Mux/45
  "IW{1,2}(45,:)'"/1 -> dotprod45/1
  dotprod44/1 -> Mux/44
  "IW{1,2}(44,:)'"/1 -> dotprod44/1
  dotprod43/1 -> Mux/43
  "IW{1,2}(43,:)'"/1 -> dotprod43/1
  dotprod42/1 -> Mux/42
  "IW{1,2}(42,:)'"/1 -> dotprod42/1
  dotprod41/1 -> Mux/41
  "IW{1,2}(41,:)'"/1 -> dotprod41/1
  dotprod40/1 -> Mux/40
  "IW{1,2}(40,:)'"/1 -> dotprod40/1
  dotprod39/1 -> Mux/39
  "IW{1,2}(39,:)'"/1 -> dotprod39/1
  dotprod38/1 -> Mux/38
  "IW{1,2}(38,:)'"/1 -> dotprod38/1
  dotprod37/1 -> Mux/37
  "IW{1,2}(37,:)'"/1 -> dotprod37/1
  dotprod36/1 -> Mux/36
  "IW{1,2}(36,:)'"/1 -> dotprod36/1
  dotprod35/1 -> Mux/35
  "IW{1,2}(35,:)'"/1 -> dotprod35/1
  dotprod34/1 -> Mux/34
  "IW{1,2}(34,:)'"/1 -> dotprod34/1
  dotprod33/1 -> Mux/33
  "IW{1,2}(33,:)'"/1 -> dotprod33/1
  dotprod32/1 -> Mux/32
  "IW{1,2}(32,:)'"/1 -> dotprod32/1
  dotprod31/1 -> Mux/31
  "IW{1,2}(31,:)'"/1 -> dotprod31/1
  dotprod30/1 -> Mux/30
  "IW{1,2}(30,:)'"/1 -> dotprod30/1
  dotprod29/1 -> Mux/29
  "IW{1,2}(29,:)'"/1 -> dotprod29/1
  dotprod28/1 -> Mux/28
  "IW{1,2}(28,:)'"/1 -> dotprod28/1
  dotprod27/1 -> Mux/27
  "IW{1,2}(27,:)'"/1 -> dotprod27/1
  dotprod26/1 -> Mux/26
  "IW{1,2}(26,:)'"/1 -> dotprod26/1
  dotprod25/1 -> Mux/25
  "IW{1,2}(25,:)'"/1 -> dotprod25/1
  dotprod24/1 -> Mux/24
  "IW{1,2}(24,:)'"/1 -> dotprod24/1
  dotprod23/1 -> Mux/23
  "IW{1,2}(23,:)'"/1 -> dotprod23/1
  dotprod22/1 -> Mux/22
  "IW{1,2}(22,:)'"/1 -> dotprod22/1
  dotprod21/1 -> Mux/21
  "IW{1,2}(21,:)'"/1 -> dotprod21/1
  dotprod20/1 -> Mux/20
  "IW{1,2}(20,:)'"/1 -> dotprod20/1
  dotprod19/1 -> Mux/19
  "IW{1,2}(19,:)'"/1 -> dotprod19/1
  dotprod18/1 -> Mux/18
  "IW{1,2}(18,:)'"/1 -> dotprod18/1
  dotprod17/1 -> Mux/17
  "IW{1,2}(17,:)'"/1 -> dotprod17/1
  dotprod16/1 -> Mux/16
  "IW{1,2}(16,:)'"/1 -> dotprod16/1
  dotprod15/1 -> Mux/15
  "IW{1,2}(15,:)'"/1 -> dotprod15/1
  dotprod14/1 -> Mux/14
  "IW{1,2}(14,:)'"/1 -> dotprod14/1
  dotprod13/1 -> Mux/13
  "IW{1,2}(13,:)'"/1 -> dotprod13/1
  dotprod12/1 -> Mux/12
  "IW{1,2}(12,:)'"/1 -> dotprod12/1
  dotprod11/1 -> Mux/11
  "IW{1,2}(11,:)'"/1 -> dotprod11/1
  dotprod10/1 -> Mux/10
  "IW{1,2}(10,:)'"/1 -> dotprod10/1
  dotprod9/1 -> Mux/9
  "IW{1,2}(9,:)'"/1 -> dotprod9/1
  dotprod8/1 -> Mux/8
  "IW{1,2}(8,:)'"/1 -> dotprod8/1
  dotprod7/1 -> Mux/7
  "IW{1,2}(7,:)'"/1 -> dotprod7/1
  dotprod6/1 -> Mux/6
  "IW{1,2}(6,:)'"/1 -> dotprod6/1
  dotprod5/1 -> Mux/5
  "IW{1,2}(5,:)'"/1 -> dotprod5/1
  dotprod4/1 -> Mux/4
  "IW{1,2}(4,:)'"/1 -> dotprod4/1
  dotprod3/1 -> Mux/3
  "IW{1,2}(3,:)'"/1 -> dotprod3/1
  dotprod2/1 -> Mux/2
  "IW{1,2}(2,:)'"/1 -> dotprod2/1
  dotprod1/1 -> Mux/1
  "pd{1,2}"/1 -> dotprod125/2, dotprod124/2, dotprod123/2, dotprod122/2, dotprod121/2, dotprod120/2, dotprod119/2, dotprod118/2, dotprod117/2, dotprod116/2, dotprod115/2, dotprod114/2, dotprod113/2, dotprod112/2, dotprod111/2, dotprod110/2, dotprod109/2, dotprod108/2, dotprod107/2, dotprod106/2, dotprod105/2, dotprod104/2, dotprod103/2, dotprod102/2, dotprod101/2, dotprod100/2, dotprod99/2, dotprod98/2, dotprod97/2, dotprod96/2, dotprod95/2, dotprod94/2, dotprod93/2, dotprod92/2, dotprod91/2, dotprod90/2, dotprod89/2, dotprod88/2, dotprod87/2, dotprod86/2, dotprod85/2, dotprod84/2, dotprod83/2, dotprod82/2, dotprod81/2, dotprod80/2, dotprod79/2, dotprod78/2, dotprod77/2, dotprod76/2, dotprod75/2, dotprod74/2, dotprod73/2, dotprod72/2, dotprod71/2, dotprod70/2, dotprod69/2, dotprod68/2, dotprod67/2, dotprod66/2, dotprod65/2, dotprod64/2, dotprod63/2, dotprod62/2, dotprod61/2, dotprod60/2, dotprod59/2, dotprod58/2, dotprod57/2, dotprod56/2, dotprod55/2, dotprod54/2, dotprod53/2, dotprod52/2, dotprod51/2, dotprod50/2, dotprod49/2, dotprod48/2, dotprod47/2, dotprod46/2, dotprod45/2, dotprod44/2, dotprod43/2, dotprod42/2, dotprod41/2, dotprod40/2, dotprod39/2, dotprod38/2, dotprod37/2, dotprod36/2, dotprod35/2, dotprod34/2, dotprod33/2, dotprod32/2, dotprod31/2, dotprod30/2, dotprod29/2, dotprod28/2, dotprod27/2, dotprod26/2, dotprod25/2, dotprod24/2, dotprod23/2, dotprod22/2, dotprod21/2, dotprod20/2, dotprod19/2, dotprod18/2, dotprod17/2, dotprod16/2, dotprod15/2, dotprod14/2, dotprod13/2, dotprod12/2, dotprod11/2, dotprod10/2, dotprod9/2, dotprod8/2, dotprod7/2, dotprod6/2, dotprod5/2, dotprod4/2, dotprod3/2, dotprod2/2, dotprod1/2
  "IW{1,2}(1,:)'"/1 -> dotprod1/1
